simulink model "d_024"  (Simulink 5.1)
settings: Solver=ode45  StartTime=0.0  StopTime=10.0  RelTol=1e-3
libraries: fm_lib x37
settings Model: Creator=fmilano  LastModifiedBy=fmilano  ExtModeAutoUpdateStatusClock=off  SignalLoggingName=logsout  BooleanDataType=on  RTWOptions="-aEnforceIntegerDowncast=1 -aFoldNonRolledExpr=1 -aInlineInvariantSignals=1 -aInlineParameters=0 -aLocalBlockOutputs=1 -aRollThreshold=5 -aZeroInternalMemoryAtStartup=1 -aZeroExternalMemoryAtStartup=1 -aInitFltsAndDblsToZero=1 -aForceBlockIOInitOptimize=0 -aGenerateReport=0 -aGenCodeOnly=0 -aRTWVerbose=1 -aIncludeHyperlinkInReport=0 -aLaunchReport=0 -aGenerateTraceInfo=0  -aForceParamTrailComments=0 -aGenerateComments=1 -aIgnoreCustomStorageClasses=1 -aIncHierarchyInIds=0 -aMaxRTWIdLen=31 -aShowEliminatedStatements=0 -aIncDataTypeInIds=0 -aInsertBlockDesc=0 -aIgnoreTestpoints=0 -aSimulinkBlockComments=1 -aInlinedPrmAccess=\"Literals\"  -aSuppressErrorStatus=0 -aModelReferenceCompliant=1 -aParenthesesLevel=\"Nominal\" -aModelStepFunctionPrototypeControlCompliant=0 -aPortableWordSizes=0 -aParMdlRefBuildCompliant=1 -aSupportNonInlinedSFcns=1 -aSupportContinuousTime=1 -aSupportComplex=1 -aSupportNonFinite=1 -aSupportAbsoluteTime=1 -aMultiwordLength=2048 -aTargetPreCompLibLocation=\"\" -aTargetLibSuffix=\"\" -aTargetFunctionLibrary=\"ANSI_C\" -aTargetFcnLib=\"ansi_tfl_tmw.mat\" -aMultiInstanceERTCode=0 -aLogVarNameModifier=\"rt_\" -aERTFirstTimeCompliant=0 -aIsPILTarget=0 -aCombineOutputUpdateFcns=0 -aGenerateASAP2=0 -aGenerateClassInterface=0 -aGenerateTestInterfaces=0 -aGenerateSampleERTMain=0 -aGenerateFullHeader=1 -aUtilityFuncGeneration=\"Auto\" -aIncludeFileDelimiter=\"Auto\" -aIncludeMdlTerminateFcn=1 -aPurelyIntegerCode=0 -aAutosarCompliant=0 -aERTCustomFileBanners=0 -aRTWCAPIStates=0 -aRTWCAPIParams=0 -aRTWCAPISignals=0 -aMatFileLogging=1 -aCompOptLevelCompliant=0 -aCPPClassGenCompliant=0 -aExtModeIntrfLevel=\"Level1\" -aExtModeMexFile=\"ext_comm\" -aExtModeTransport=0 -aExtModeStaticAllocSize=1000000 -aExtModeTesting=0 -aExtModeStaticAlloc=0 -aExtMode=0 -aERTMultiwordLength=256 -aERTMultiwordTypeDef=\"System defined\"  -aGenerateTraceInfo=0 -aGenerateTraceInfo=0 -aGenerateTraceInfo=0 -aGenerateTraceInfo=0 -aPrefixModelToSubsysFcnNames=1"

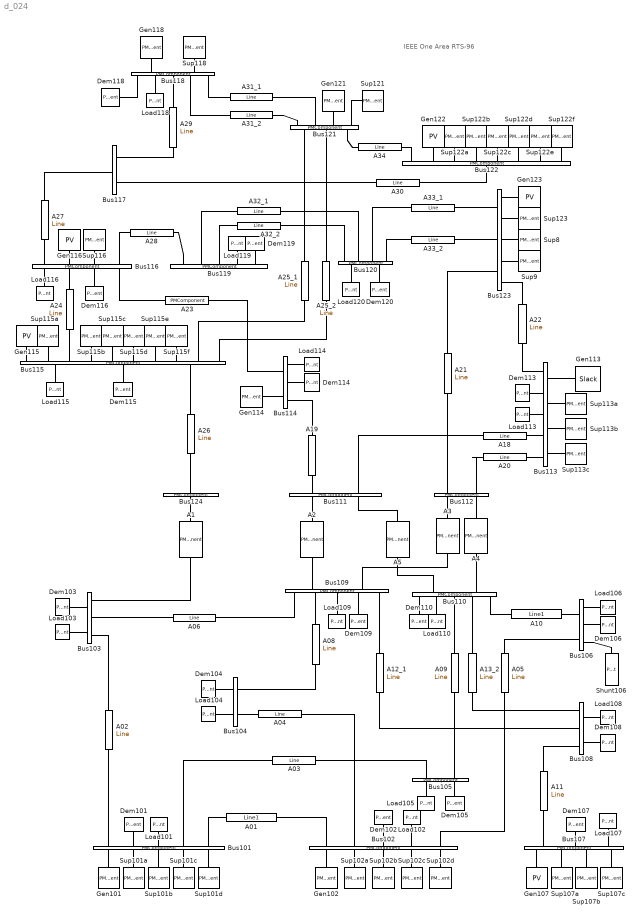
== system d_024 ==
  note: IEEE One Area RTS-96
  A01 : fm_lib/Power Flow/Line1  Tag=PSATblock  Description=Power Flow  PhysicalDomain=psatdomain  SubClassName=unknown  LeftPortType=p1  RightPortType=p1  LConnTagsString=__newl0  RConnTagsString=__newr0  p3_4_5q="[100  138  60]"  p6q=0  p8q=0.0026  p9q=0.0139  p10q=0.4611  p13_14_15q="[1.93  0.0  2.00]"  p16q=on
  A02 : fm_lib/Power Flow/Line  Tag=PSATblock  Description=Power Flow  Orientation=up  PhysicalDomain=psatdomain  SubClassName=unknown  LeftPortType=p1  RightPortType=p1  LConnTagsString=__newl0  RConnTagsString=__newr0  p3_4_5q="[100  138  60]"  p6q=0  p8q=0.0546  p9q=0.2112  p10q=0.0572  p13_14_15q="[2.08  0.0  2.20]"  p16q=on
  A03 : fm_lib/Power Flow/Line  Tag=PSATblock  Description=Power Flow  PhysicalDomain=psatdomain  SubClassName=unknown  LeftPortType=p1  RightPortType=p1  LConnTagsString=__newl0  RConnTagsString=__newr0  p3_4_5q="[100  138  60]"  p6q=0  p8q=0.0218  p9q=0.0845  p10q=0.0229  p13_14_15q="[2.08  0.0  2.20]"  p16q=on
  A04 : fm_lib/Power Flow/Line  Tag=PSATblock  Description=Power Flow  Orientation=left  PhysicalDomain=psatdomain  SubClassName=unknown  LeftPortType=p1  RightPortType=p1  LConnTagsString=__newl0  RConnTagsString=__newr0  p3_4_5q="[100  138  60]"  p6q=0  p8q=0.0328  p9q=0.1267  p10q=0.0343  p13_14_15q="[2.08  0.0  2.20]"  p16q=on
  A05 : fm_lib/Power Flow/Line  Tag=PSATblock  Description=Power Flow  Orientation=up  PhysicalDomain=psatdomain  SubClassName=unknown  LeftPortType=p1  RightPortType=p1  LConnTagsString=__newl0  RConnTagsString=__newr0  p3_4_5q="[100  138  60]"  p6q=0  p8q=0.0497  p9q=0.192  p10q=0.052  p13_14_15q="[2.08  0.0  2.20]"  p16q=on
  A06 : fm_lib/Power Flow/Line  Tag=PSATblock  Description=Power Flow  Orientation=left  PhysicalDomain=psatdomain  SubClassName=unknown  LeftPortType=p1  RightPortType=p1  LConnTagsString=__newl0  RConnTagsString=__newr0  p3_4_5q="[100  138  60]"  p6q=0  p8q=0.0308  p9q=0.119  p10q=0.0322  p13_14_15q="[2.08  0.0  2.20]"  p16q=on
  A08 : fm_lib/Power Flow/Line  Tag=PSATblock  Description=Power Flow  Orientation=down  PhysicalDomain=psatdomain  SubClassName=unknown  LeftPortType=p1  RightPortType=p1  LConnTagsString=__newl0  RConnTagsString=__newr0  p3_4_5q="[100  138  60]"  p6q=0  p8q=0.0268  p9q=0.1037  p10q=0.0281  p13_14_15q="[2.08  0.0  2.20]"  p16q=on
  A09 : fm_lib/Power Flow/Line  Tag=PSATblock  Description=Power Flow  Orientation=down  PhysicalDomain=psatdomain  SubClassName=unknown  LeftPortType=p1  RightPortType=p1  LConnTagsString=__newl0  RConnTagsString=__newr0  p3_4_5q="[100  138  60]"  p6q=0  p8q=0.0228  p9q=0.0883  p10q=0.0239  p13_14_15q="[2.08  0.0  2.20]"  p16q=on
  A1 : PMComponent  Tag=PSATblock  Description=Power Flow  Orientation=up  PhysicalDomain=psatdomain  LeftPortType=p1  RightPortType=p1  LConnTagsString=__newl0  RConnTagsString=__newr0  mask(Line){p3_4_5q=[100  138  60], p7q=138/230, p8q=0.0023, p9q=0.0839, p11q=1.015, p13_14_15q=[5.10  0.0  6.00], p16q=on}
      mask prompts: p3_4_5q "Power, Voltage and Frequency Ratings [MVA, kV, Hz]"; p7q "Primary and secondary voltage ratio [kV/kV]"; p8q "Resistance [p.u.]"; p9q "Reactance [p.u.]"; p11q "Fixed tap ratio [p.u./p.u.]"; p13_14_15q "Imax, Pmax and Smax  [p.u., p.u., p.u.]"; p16q "Connected"
      mask help: This block defines a transformer with constant tap ratio.
      mask init:
      | [x,y] = fm_draw('circle');
      | [x2,y2] = fm_draw('2');
      mask CallbackString: ||||||fm_block
      mask Display:
      | plot(x,y,x+1.4,y,[-1 -1.3],[0 0],[2.4 2.7],[0 0])
      | color('green')
      | plot([-0.8 0.7],[-1.2 1.2],[0.5 0.7],[1.1 1.2],[0.7 0.7],[1.0 1.2])
      | plot(1.5+0.65*x2,0.65*y2)
  A10 : fm_lib/Power Flow/Line1  Tag=PSATblock  Description=Power Flow  PhysicalDomain=psatdomain  SubClassName=unknown  LeftPortType=p1  RightPortType=p1  LConnTagsString=__newl0  RConnTagsString=__newr0  p3_4_5q="[100  138  60]"  p6q=0  p8q=0.0139  p9q=0.0605  p10q=2.459  p13_14_15q="[1.93  0.0  2.00]"  p16q=on
  A11 : fm_lib/Power Flow/Line  Tag=PSATblock  Description=Power Flow  Orientation=up  PhysicalDomain=psatdomain  SubClassName=unknown  LeftPortType=p1  RightPortType=p1  LConnTagsString=__newl0  RConnTagsString=__newr0  p3_4_5q="[100  138  60]"  p6q=0  p8q=0.0159  p9q=0.0614  p10q=0.0166  p13_14_15q="[2.08  0.0  2.20]"  p16q=on
  A12_1 : fm_lib/Power Flow/Line  Tag=PSATblock  Description=Power Flow  Orientation=down  PhysicalDomain=psatdomain  SubClassName=unknown  LeftPortType=p1  RightPortType=p1  LConnTagsString=__newl0  RConnTagsString=__newr0  p3_4_5q="[100  138  60]"  p6q=0  p8q=0.0427  p9q=0.1651  p10q=0.0447  p13_14_15q="[2.08  0.0  2.20]"  p16q=on
  A13_2 : fm_lib/Power Flow/Line  Tag=PSATblock  Description=Power Flow  Orientation=down  PhysicalDomain=psatdomain  SubClassName=unknown  LeftPortType=p1  RightPortType=p1  LConnTagsString=__newl0  RConnTagsString=__newr0  p3_4_5q="[100  138  60]"  p6q=0  p8q=0.0427  p9q=0.1651  p10q=0.0447  p13_14_15q="[2.08  0.0  2.20]"  p16q=on
  A18 : fm_lib/Power Flow/Line  Tag=PSATblock  Description=Power Flow  Orientation=left  PhysicalDomain=psatdomain  SubClassName=unknown  LeftPortType=p1  RightPortType=p1  LConnTagsString=__newl0  RConnTagsString=__newr0  p3_4_5q="[100  230  60]"  p6q=0  p8q=0.006  p9q=0.048  p10q=0.100  p13_14_15q="[6.00  0.0  6.25]"  p16q=on
  A19 : PMComponent  Tag=PSATblock  Description=Power Flow  Orientation=down  PhysicalDomain=psatdomain  LeftPortType=p1  RightPortType=p1  LConnTagsString=__newl0  RConnTagsString=__newr0  mask(Line){p3_4_5q=[100  230  60], p6q=0, p8q=0.0054, p9q=0.0418, p10q=0.0879, p13_14_15q=[6.00  0.0  6.25], p16q=on}
      mask prompts: p3_4_5q "Power, Voltage and Frequency Ratings [MVA, kV, Hz]"; p6q "Length of line [km] (0 for p.u. parameters)"; p8q "Resistance [p.u. (Ohms/km)]"; p9q "Reactance [p.u. (H/km)]"; p10q "Susceptance [p.u. (F/km)]"; p13_14_15q "Imax, Pmax and Smax [p.u., p.u., p.u.]"; p16q "Connected"
      mask help: This block defines a pi model for a tree phase line.
      mask init:
      | [xp,yp] = fm_draw('pi');
      mask CallbackString: ||||||fm_block
      mask Display:
      | plot([-1  1  1 -1 -1],[-0.2 -0.2 0.2 0.2 -0.2])
      | color('blue')
      | plot(0.35*xp,0.2*yp)
  A2 : PMComponent  Tag=PSATblock  Description=Power Flow  Orientation=up  PhysicalDomain=psatdomain  LeftPortType=p1  RightPortType=p1  LConnTagsString=__newl0  RConnTagsString=__newr0  mask(Line){p3_4_5q=[100  138  60], p7q=138/230, p8q=0.0023, p9q=0.0839, p11q=1.03, p13_14_15q=[5.10  0.0  6.00], p16q=on}
      mask prompts: p3_4_5q "Power, Voltage and Frequency Ratings [MVA, kV, Hz]"; p7q "Primary and secondary voltage ratio [kV/kV]"; p8q "Resistance [p.u.]"; p9q "Reactance [p.u.]"; p11q "Fixed tap ratio [p.u./p.u.]"; p13_14_15q "Imax, Pmax and Smax  [p.u., p.u., p.u.]"; p16q "Connected"
      mask help: This block defines a transformer with constant tap ratio.
      mask init:
      | [x,y] = fm_draw('circle');
      | [x2,y2] = fm_draw('2');
      mask CallbackString: ||||||fm_block
      mask Display:
      | plot(x,y,x+1.4,y,[-1 -1.3],[0 0],[2.4 2.7],[0 0])
      | color('green')
      | plot([-0.8 0.7],[-1.2 1.2],[0.5 0.7],[1.1 1.2],[0.7 0.7],[1.0 1.2])
      | plot(1.5+0.65*x2,0.65*y2)
  A20 : fm_lib/Power Flow/Line  Tag=PSATblock  Description=Power Flow  Orientation=left  PhysicalDomain=psatdomain  SubClassName=unknown  LeftPortType=p1  RightPortType=p1  LConnTagsString=__newl0  RConnTagsString=__newr0  p3_4_5q="[100  230  60]"  p6q=0  p8q=0.006  p9q=0.048  p10q=0.100  p13_14_15q="[6.00  0.0  6.25]"  p16q=on
  A21 : fm_lib/Power Flow/Line  Tag=PSATblock  Description=Power Flow  Orientation=down  PhysicalDomain=psatdomain  SubClassName=unknown  LeftPortType=p1  RightPortType=p1  LConnTagsString=__newl0  RConnTagsString=__newr0  p3_4_5q="[100  230  60]"  p6q=0  p8q=0.0124  p9q=0.0966  p10q=0.203  p13_14_15q="[6.00  0.0  6.25]"  p16q=on
  A22 : fm_lib/Power Flow/Line  Tag=PSATblock  Description=Power Flow  Orientation=up  PhysicalDomain=psatdomain  SubClassName=unknown  LeftPortType=p1  RightPortType=p1  LConnTagsString=__newl0  RConnTagsString=__newr0  p3_4_5q="[100  230  60]"  p6q=0  p8q=0.0111  p9q=0.0865  p10q=0.1818  p13_14_15q="[6.00  0.0  6.25]"  p16q=on
  A23 : PMComponent  Tag=PSATblock  Description=Power Flow  PhysicalDomain=psatdomain  LeftPortType=p1  RightPortType=p1  LConnTagsString=__newl0  RConnTagsString=__newr0  mask(Line){p3_4_5q=[100  230  60], p6q=0, p8q=0.005, p9q=0.0589, p10q=0.0818, p13_14_15q=[6.00  0.0  6.25], p16q=on}
      mask prompts: p3_4_5q "Power, Voltage and Frequency Ratings [MVA, kV, Hz]"; p6q "Length of line [km] (0 for p.u. parameters)"; p8q "Resistance [p.u. (Ohms/km)]"; p9q "Reactance [p.u. (H/km)]"; p10q "Susceptance [p.u. (F/km)]"; p13_14_15q "Imax, Pmax and Smax [p.u., p.u., p.u.]"; p16q "Connected"
      mask help: This block defines a pi model for a tree phase line.
      mask init:
      | [xp,yp] = fm_draw('pi');
      mask CallbackString: ||||||fm_block
      mask Display:
      | plot([-1  1  1 -1 -1],[-0.2 -0.2 0.2 0.2 -0.2])
      | color('blue')
      | plot(0.35*xp,0.2*yp)
  A24 : fm_lib/Power Flow/Line  Tag=PSATblock  Description=Power Flow  Orientation=down  PhysicalDomain=psatdomain  SubClassName=unknown  LeftPortType=p1  RightPortType=p1  LConnTagsString=__newl0  RConnTagsString=__newr0  p3_4_5q="[100  230  60]"  p6q=0  p8q=0.0022  p9q=0.0173  p10q=0.0364  p13_14_15q="[6.00  0.0  6.25]"  p16q=on
  A25_1 : fm_lib/Power Flow/Line  Tag=PSATblock  Description=Power Flow  Orientation=down  PhysicalDomain=psatdomain  SubClassName=unknown  LeftPortType=p1  RightPortType=p1  LConnTagsString=__newl0  RConnTagsString=__newr0  p3_4_5q="[100  230  60]"  p6q=0  p8q=0.0063  p9q=0.049  p10q=0.103  p13_14_15q="[6.00  0.0  6.25]"  p16q=on
  A25_2 : fm_lib/Power Flow/Line  Tag=PSATblock  Description=Power Flow  Orientation=down  PhysicalDomain=psatdomain  SubClassName=unknown  LeftPortType=p1  RightPortType=p1  LConnTagsString=__newl0  RConnTagsString=__newr0  p3_4_5q="[100  230  60]"  p6q=0  p8q=0.0063  p9q=0.049  p10q=0.103  p13_14_15q="[6.00  0.0  6.25]"  p16q=on
  A26 : fm_lib/Power Flow/Line  Tag=PSATblock  Description=Power Flow  Orientation=down  PhysicalDomain=psatdomain  SubClassName=unknown  LeftPortType=p1  RightPortType=p1  LConnTagsString=__newl0  RConnTagsString=__newr0  p3_4_5q="[100  230  60]"  p6q=0  p8q=0.0067  p9q=0.0519  p10q=0.1091  p13_14_15q="[6.00  0.0  6.25]"  p16q=on
  A27 : fm_lib/Power Flow/Line  Tag=PSATblock  Description=Power Flow  Orientation=down  PhysicalDomain=psatdomain  SubClassName=unknown  LeftPortType=p1  RightPortType=p1  LConnTagsString=__newl0  RConnTagsString=__newr0  p3_4_5q="[100  230  60]"  p6q=0  p8q=0.003  p9q=0.0259  p10q=0.0545  p13_14_15q="[6.00  0.0  6.25]"  p16q=on
  A28 : fm_lib/Power Flow/Line  Tag=PSATblock  Description=Power Flow  Orientation=left  PhysicalDomain=psatdomain  SubClassName=unknown  LeftPortType=p1  RightPortType=p1  LConnTagsString=__newl0  RConnTagsString=__newr0  p3_4_5q="[100  230  60]"  p6q=0  p8q=0.003  p9q=0.0231  p10q=0.0485  p13_14_15q="[6.00  0.0  6.25]"  p16q=on
  A29 : fm_lib/Power Flow/Line  Tag=PSATblock  Description=Power Flow  Orientation=down  PhysicalDomain=psatdomain  SubClassName=unknown  LeftPortType=p1  RightPortType=p1  LConnTagsString=__newl0  RConnTagsString=__newr0  p3_4_5q="[100  230  60]"  p6q=0  p8q=0.0018  p9q=0.0144  p10q=0.0303  p13_14_15q="[6.00  0.0  6.25]"  p16q=on
  A3 : PMComponent  Tag=PSATblock  Description=Power Flow  Orientation=up  PhysicalDomain=psatdomain  LeftPortType=p1  RightPortType=p1  LConnTagsString=__newl0  RConnTagsString=__newr0  mask(Line){p3_4_5q=[100  138  60], p7q=138/230, p8q=0.0023, p9q=0.0839, p11q=1.03, p13_14_15q=[5.10  0.0  6.00], p16q=on}
      mask prompts: p3_4_5q "Power, Voltage and Frequency Ratings [MVA, kV, Hz]"; p7q "Primary and secondary voltage ratio [kV/kV]"; p8q "Resistance [p.u.]"; p9q "Reactance [p.u.]"; p11q "Fixed tap ratio [p.u./p.u.]"; p13_14_15q "Imax, Pmax and Smax  [p.u., p.u., p.u.]"; p16q "Connected"
      mask help: This block defines a transformer with constant tap ratio.
      mask init:
      | [x,y] = fm_draw('circle');
      | [x2,y2] = fm_draw('2');
      mask CallbackString: ||||||fm_block
      mask Display:
      | plot(x,y,x+1.4,y,[-1 -1.3],[0 0],[2.4 2.7],[0 0])
      | color('green')
      | plot([-0.8 0.7],[-1.2 1.2],[0.5 0.7],[1.1 1.2],[0.7 0.7],[1.0 1.2])
      | plot(1.5+0.65*x2,0.65*y2)
  A30 : fm_lib/Power Flow/Line  Tag=PSATblock  Description=Power Flow  Orientation=left  PhysicalDomain=psatdomain  SubClassName=unknown  LeftPortType=p1  RightPortType=p1  LConnTagsString=__newl0  RConnTagsString=__newr0  p3_4_5q="[100  230  60]"  p6q=0  p8q=0.0135  p9q=0.1053  p10q=0.2212  p13_14_15q="[6.00  0.0  6.25]"  p16q=on
  A31_1 : fm_lib/Power Flow/Line  Tag=PSATblock  Description=Power Flow  PhysicalDomain=psatdomain  SubClassName=unknown  LeftPortType=p1  RightPortType=p1  LConnTagsString=__newl0  RConnTagsString=__newr0  p3_4_5q="[100  230  60]"  p6q=0  p8q=0.0033  p9q=0.0269  p10q=0.0545  p13_14_15q="[6.00  0.0  6.25]"  p16q=on
  A31_2 : fm_lib/Power Flow/Line  Tag=PSATblock  Description=Power Flow  PhysicalDomain=psatdomain  SubClassName=unknown  LeftPortType=p1  RightPortType=p1  LConnTagsString=__newl0  RConnTagsString=__newr0  p3_4_5q="[100  230  60]"  p6q=0  p8q=0.0033  p9q=0.0269  p10q=0.0545  p13_14_15q="[6.00  0.0  6.25]"  p16q=on
  A32_1 : fm_lib/Power Flow/Line  Tag=PSATblock  Description=Power Flow  PhysicalDomain=psatdomain  SubClassName=unknown  LeftPortType=p1  RightPortType=p1  LConnTagsString=__newl0  RConnTagsString=__newr0  p3_4_5q="[100  230  60]"  p6q=0  p8q=0.0051  p9q=0.0396  p10q=0.0833  p13_14_15q="[6.00  0.0  6.25]"  p16q=on
  A32_2 : fm_lib/Power Flow/Line  Tag=PSATblock  Description=Power Flow  PhysicalDomain=psatdomain  SubClassName=unknown  LeftPortType=p1  RightPortType=p1  LConnTagsString=__newl0  RConnTagsString=__newr0  p3_4_5q="[100  230  60]"  p6q=0  p8q=0.0051  p9q=0.0396  p10q=0.0833  p13_14_15q="[6.00  0.0  6.25]"  p16q=on
  A33_1 : fm_lib/Power Flow/Line  Tag=PSATblock  Description=Power Flow  Orientation=left  PhysicalDomain=psatdomain  SubClassName=unknown  LeftPortType=p1  RightPortType=p1  LConnTagsString=__newl0  RConnTagsString=__newr0  p3_4_5q="[100  230  60]"  p6q=0  p8q=0.0028  p9q=0.0216  p10q=0.0455  p13_14_15q="[6.00  0.0  6.25]"  p16q=on
  A33_2 : fm_lib/Power Flow/Line  Tag=PSATblock  Description=Power Flow  Orientation=left  PhysicalDomain=psatdomain  SubClassName=unknown  LeftPortType=p1  RightPortType=p1  LConnTagsString=__newl0  RConnTagsString=__newr0  p3_4_5q="[100  230  60]"  p6q=0  p8q=0.0028  p9q=0.0216  p10q=0.0455  p13_14_15q="[6.00  0.0  6.25]"  p16q=on
  A34 : fm_lib/Power Flow/Line  Tag=PSATblock  Description=Power Flow  PhysicalDomain=psatdomain  SubClassName=unknown  LeftPortType=p1  RightPortType=p1  LConnTagsString=__newl0  RConnTagsString=__newr0  p3_4_5q="[100  230  60]"  p6q=0  p8q=0.0087  p9q=0.0678  p10q=0.1424  p13_14_15q="[6.00  0.0  6.25]"  p16q=on
  A4 : PMComponent  Tag=PSATblock  Description=Power Flow  Orientation=up  PhysicalDomain=psatdomain  LeftPortType=p1  RightPortType=p1  LConnTagsString=__newl0  RConnTagsString=__newr0  mask(Line){p3_4_5q=[100  138  60], p7q=138/230, p8q=0.0023, p9q=0.0839, p11q=1.015, p13_14_15q=[5.10  0.0  6.00], p16q=on}
      mask prompts: p3_4_5q "Power, Voltage and Frequency Ratings [MVA, kV, Hz]"; p7q "Primary and secondary voltage ratio [kV/kV]"; p8q "Resistance [p.u.]"; p9q "Reactance [p.u.]"; p11q "Fixed tap ratio [p.u./p.u.]"; p13_14_15q "Imax, Pmax and Smax  [p.u., p.u., p.u.]"; p16q "Connected"
      mask help: This block defines a transformer with constant tap ratio.
      mask init:
      | [x,y] = fm_draw('circle');
      | [x2,y2] = fm_draw('2');
      mask CallbackString: ||||||fm_block
      mask Display:
      | plot(x,y,x+1.4,y,[-1 -1.3],[0 0],[2.4 2.7],[0 0])
      | color('green')
      | plot([-0.8 0.7],[-1.2 1.2],[0.5 0.7],[1.1 1.2],[0.7 0.7],[1.0 1.2])
      | plot(1.5+0.65*x2,0.65*y2)
  A5 : PMComponent  Tag=PSATblock  Description=Power Flow  Orientation=up  PhysicalDomain=psatdomain  LeftPortType=p1  RightPortType=p1  LConnTagsString=__newl0  RConnTagsString=__newr0  mask(Line){p3_4_5q=[100  138  60], p7q=138/230, p8q=0.0023, p9q=0.0839, p11q=1.015, p13_14_15q=[5.10  0.0  6.00], p16q=on}
      mask prompts: p3_4_5q "Power, Voltage and Frequency Ratings [MVA, kV, Hz]"; p7q "Primary and secondary voltage ratio [kV/kV]"; p8q "Resistance [p.u.]"; p9q "Reactance [p.u.]"; p11q "Fixed tap ratio [p.u./p.u.]"; p13_14_15q "Imax, Pmax and Smax  [p.u., p.u., p.u.]"; p16q "Connected"
      mask help: This block defines a transformer with constant tap ratio.
      mask init:
      | [x,y] = fm_draw('circle');
      | [x2,y2] = fm_draw('2');
      mask CallbackString: ||||||fm_block
      mask Display:
      | plot(x,y,x+1.4,y,[-1 -1.3],[0 0],[2.4 2.7],[0 0])
      | color('green')
      | plot([-0.8 0.7],[-1.2 1.2],[0.5 0.7],[1.1 1.2],[0.7 0.7],[1.0 1.2])
      | plot(1.5+0.65*x2,0.65*y2)
  Bus101 : PMComponent  Tag=PSATblock  Description=Connection  Orientation=up  PhysicalDomain=psatdomain  LeftPortType=p1  RightPortType=p1  LConnTagsString=__newl0|__newl1|__newl2|__newl3|__newl4  RConnTagsString=__newr0|__newr1|__newr2|__newr3|__newr4  mask(Bus){in=5, out=5, p2q=138, p3_4q=[1.00  0.00], p5q=2, p6q=1}
      mask prompts: in "Number of inputs:"; out "Number of outputs:"; p2q "Voltage Rating [kV]"; p3_4q "Voltage initial guess [p.u.  rad]"; p5q "Area number"; p6q "Region number"
      mask help: Bus block.
      mask init:
      | fm_inout
      mask CallbackString: ||||fm_block|
      mask Display: plot([0 1 1 0 0],[0 0 1 1 0])
  Bus102 : PMComponent  Tag=PSATblock  Description=Connection  Orientation=up  PhysicalDomain=psatdomain  LeftPortType=p1  RightPortType=p1  LConnTagsString=__newl0|__newl1|__newl2|__newl3|__newl4  RConnTagsString=__newr0|__newr1|__newr2|__newr3|__newr4  mask(Bus){in=5, out=5, p2q=138, p3_4q=[1.00  0.00], p5q=2, p6q=1}
      mask prompts: in "Number of inputs:"; out "Number of outputs:"; p2q "Voltage Rating [kV]"; p3_4q "Voltage initial guess [p.u.  rad]"; p5q "Area number"; p6q "Region number"
      mask help: Bus block.
      mask init:
      | fm_inout
      mask CallbackString: ||||fm_block|
      mask Display: plot([0 1 1 0 0],[0 0 1 1 0])
  Bus103 : PMComponent  Tag=PSATblock  Description=Connection  Orientation=left  PhysicalDomain=psatdomain  LeftPortType=p1  RightPortType=p1  LConnTagsString=__newl0|__newl1|__newl2  RConnTagsString=__newr0|__newr1  mask(Bus){in=3, out=2, p2q=138, p3_4q=[1.00   0.00], p5q=2, p6q=1}
      mask prompts: in "Number of inputs:"; out "Number of outputs:"; p2q "Voltage Rating [kV]"; p3_4q "Voltage initial guess [p.u.  rad]"; p5q "Area number"; p6q "Region number"
      mask help: Bus block.
      mask init:
      | fm_inout
      mask CallbackString: ||||fm_block|
      mask Display: plot([0 1 1 0 0],[0 0 1 1 0])
  Bus104 : PMComponent  Tag=PSATblock  Description=Connection  Orientation=left  PhysicalDomain=psatdomain  LeftPortType=p1  RightPortType=p1  LConnTagsString=__newl0|__newl1  RConnTagsString=__newr0|__newr1  mask(Bus){in=2, out=2, p2q=138, p3_4q=[1.00   0.00], p5q=2, p6q=1}
      mask prompts: in "Number of inputs:"; out "Number of outputs:"; p2q "Voltage Rating [kV]"; p3_4q "Voltage initial guess [p.u.  rad]"; p5q "Area number"; p6q "Region number"
      mask help: Bus block.
      mask init:
      | fm_inout
      mask CallbackString: ||||fm_block|
      mask Display: plot([0 1 1 0 0],[0 0 1 1 0])
  Bus105 : PMComponent  Tag=PSATblock  Description=Connection  Orientation=down  PhysicalDomain=psatdomain  LeftPortType=p1  RightPortType=p1  LConnTagsString=__newl0|__newl1  RConnTagsString=__newr0|__newr1  mask(Bus){in=2, out=2, p2q=138, p3_4q=[1.00   0.00], p5q=2, p6q=1}
      mask prompts: in "Number of inputs:"; out "Number of outputs:"; p2q "Voltage Rating [kV]"; p3_4q "Voltage initial guess [p.u.  rad]"; p5q "Area number"; p6q "Region number"
      mask help: Bus block.
      mask init:
      | fm_inout
      mask CallbackString: ||||fm_block|
      mask Display: plot([0 1 1 0 0],[0 0 1 1 0])
  Bus106 : PMComponent  Tag=PSATblock  Description=Connection  PhysicalDomain=psatdomain  LeftPortType=p1  RightPortType=p1  LConnTagsString=__newl0|__newl1  RConnTagsString=__newr0|__newr1|__newr2  mask(Bus){in=2, out=3, p2q=138, p3_4q=[1.00   0.00], p5q=2, p6q=1}
      mask prompts: in "Number of inputs:"; out "Number of outputs:"; p2q "Voltage Rating [kV]"; p3_4q "Voltage initial guess [p.u.  rad]"; p5q "Area number"; p6q "Region number"
      mask help: Bus block.
      mask init:
      | fm_inout
      mask CallbackString: ||||fm_block|
      mask Display: plot([0 1 1 0 0],[0 0 1 1 0])
  Bus107 : PMComponent  Tag=PSATblock  Description=Connection  Orientation=up  PhysicalDomain=psatdomain  LeftPortType=p1  RightPortType=p1  LConnTagsString=__newl0|__newl1|__newl2|__newl3  RConnTagsString=__newr0|__newr1|__newr2  mask(Bus){in=4, out=3, p2q=138, p3_4q=[1.00  0.00], p5q=2, p6q=1}
      mask prompts: in "Number of inputs:"; out "Number of outputs:"; p2q "Voltage Rating [kV]"; p3_4q "Voltage initial guess [p.u.  rad]"; p5q "Area number"; p6q "Region number"
      mask help: Bus block.
      mask init:
      | fm_inout
      mask CallbackString: ||||fm_block|
      mask Display: plot([0 1 1 0 0],[0 0 1 1 0])
  Bus108 : PMComponent  Tag=PSATblock  Description=Connection  PhysicalDomain=psatdomain  LeftPortType=p1  RightPortType=p1  LConnTagsString=__newl0|__newl1|__newl2  RConnTagsString=__newr0|__newr1  mask(Bus){in=3, out=2, p2q=138, p3_4q=[1.00   0.00], p5q=2, p6q=1}
      mask prompts: in "Number of inputs:"; out "Number of outputs:"; p2q "Voltage Rating [kV]"; p3_4q "Voltage initial guess [p.u.  rad]"; p5q "Area number"; p6q "Region number"
      mask help: Bus block.
      mask init:
      | fm_inout
      mask CallbackString: ||||fm_block|
      mask Display: plot([0 1 1 0 0],[0 0 1 1 0])
  Bus109 : PMComponent  Tag=PSATblock  Description=Connection  Orientation=down  PhysicalDomain=psatdomain  LeftPortType=p1  RightPortType=p1  LConnTagsString=__newl0|__newl1  RConnTagsString=__newr0|__newr1|__newr2|__newr3|__newr4  mask(Bus){in=2, out=5, p2q=138, p3_4q=[1.00  0.00], p5q=2, p6q=1}
      mask prompts: in "Number of inputs:"; out "Number of outputs:"; p2q "Voltage Rating [kV]"; p3_4q "Voltage initial guess [p.u.  rad]"; p5q "Area number"; p6q "Region number"
      mask help: Bus block.
      mask init:
      | fm_inout
      mask CallbackString: ||||fm_block|
      mask Display: plot([0 1 1 0 0],[0 0 1 1 0])
  Bus110 : PMComponent  Tag=PSATblock  Description=Connection  Orientation=down  PhysicalDomain=psatdomain  LeftPortType=p1  RightPortType=p1  LConnTagsString=__newl0|__newl1  RConnTagsString=__newr0|__newr1|__newr2|__newr3|__newr4  mask(Bus){in=2, out=5, p2q=138, p3_4q=[1.00  0.00], p5q=2, p6q=1}
      mask prompts: in "Number of inputs:"; out "Number of outputs:"; p2q "Voltage Rating [kV]"; p3_4q "Voltage initial guess [p.u.  rad]"; p5q "Area number"; p6q "Region number"
      mask help: Bus block.
      mask init:
      | fm_inout
      mask CallbackString: ||||fm_block|
      mask Display: plot([0 1 1 0 0],[0 0 1 1 0])
  Bus111 : PMComponent  Tag=PSATblock  Description=Connection  Orientation=down  PhysicalDomain=psatdomain  LeftPortType=p1  RightPortType=p1  LConnTagsString=__newl0|__newl1  RConnTagsString=__newr0|__newr1  mask(Bus){in=2, out=2, p2q=230, p3_4q=[1.00  0.00], p5q=3, p6q=1}
      mask prompts: in "Number of inputs:"; out "Number of outputs:"; p2q "Voltage Rating [kV]"; p3_4q "Voltage initial guess [p.u.  rad]"; p5q "Area number"; p6q "Region number"
      mask help: Bus block.
      mask init:
      | fm_inout
      mask CallbackString: ||||fm_block|
      mask Display: plot([0 1 1 0 0],[0 0 1 1 0])
  Bus112 : PMComponent  Tag=PSATblock  Description=Connection  Orientation=down  PhysicalDomain=psatdomain  LeftPortType=p1  RightPortType=p1  LConnTagsString=__newl0|__newl1  RConnTagsString=__newr0|__newr1  mask(Bus){in=2, out=2, p2q=230, p3_4q=[1.00  0.00], p5q=3, p6q=1}
      mask prompts: in "Number of inputs:"; out "Number of outputs:"; p2q "Voltage Rating [kV]"; p3_4q "Voltage initial guess [p.u.  rad]"; p5q "Area number"; p6q "Region number"
      mask help: Bus block.
      mask init:
      | fm_inout
      mask CallbackString: ||||fm_block|
      mask Display: plot([0 1 1 0 0],[0 0 1 1 0])
  Bus113 : PMComponent  Tag=PSATblock  Description=Connection  Orientation=left  PhysicalDomain=psatdomain  LeftPortType=p1  RightPortType=p1  LConnTagsString=__newl0|__newl1|__newl2|__newl3  RConnTagsString=__newr0|__newr1|__newr2|__newr3|__newr4  mask(Bus){in=4, out=5, p2q=230, p3_4q=[1.00   0.00], p5q=3, p6q=1}
      mask prompts: in "Number of inputs:"; out "Number of outputs:"; p2q "Voltage Rating [kV]"; p3_4q "Voltage initial guess [p.u.  rad]"; p5q "Area number"; p6q "Region number"
      mask help: Bus block.
      mask init:
      | fm_inout
      mask CallbackString: ||||fm_block|
      mask Display: plot([0 1 1 0 0],[0 0 1 1 0])
  Bus114 : PMComponent  Tag=PSATblock  Description=Connection  PhysicalDomain=psatdomain  LeftPortType=p1  RightPortType=p1  LConnTagsString=__newl0|__newl1  RConnTagsString=__newr0|__newr1|__newr2  mask(Bus){in=2, out=3, p2q=230, p3_4q=[1.00   0.00], p5q=3, p6q=1}
      mask prompts: in "Number of inputs:"; out "Number of outputs:"; p2q "Voltage Rating [kV]"; p3_4q "Voltage initial guess [p.u.  rad]"; p5q "Area number"; p6q "Region number"
      mask help: Bus block.
      mask init:
      | fm_inout
      mask CallbackString: ||||fm_block|
      mask Display: plot([0 1 1 0 0],[0 0 1 1 0])
  Bus115 : PMComponent  Tag=PSATblock  Description=Connection  Orientation=down  PhysicalDomain=psatdomain  LeftPortType=p1  RightPortType=p1  LConnTagsString=__newl0|__newl1|__newl2|__newl3|__newl4|__newl5|__newl6|__newl7|__newl8|__newl9  RConnTagsString=__newr0|__newr1|__newr2  mask(Bus){in=10, out=3, p2q=230, p3_4q=[1.00  0.00], p5q=3, p6q=1}
      mask prompts: in "Number of inputs:"; out "Number of outputs:"; p2q "Voltage Rating [kV]"; p3_4q "Voltage initial guess [p.u.  rad]"; p5q "Area number"; p6q "Region number"
      mask help: Bus block.
      mask init:
      | fm_inout
      mask CallbackString: ||||fm_block|
      mask Display: plot([0 1 1 0 0],[0 0 1 1 0])
  Bus116 : PMComponent  Tag=PSATblock  Description=Connection  Orientation=down  PhysicalDomain=psatdomain  LeftPortType=p1  RightPortType=p1  LConnTagsString=__newl0|__newl1|__newl2|__newl3  RConnTagsString=__newr0|__newr1|__newr2|__newr3  mask(Bus){in=4, out=4, p2q=230, p3_4q=[1.00  0.00], p5q=3, p6q=1}
      mask prompts: in "Number of inputs:"; out "Number of outputs:"; p2q "Voltage Rating [kV]"; p3_4q "Voltage initial guess [p.u.  rad]"; p5q "Area number"; p6q "Region number"
      mask help: Bus block.
      mask init:
      | fm_inout
      mask CallbackString: ||||fm_block|
      mask Display: plot([0 1 1 0 0],[0 0 1 1 0])
  Bus117 : PMComponent  Tag=PSATblock  Description=Connection  Orientation=left  PhysicalDomain=psatdomain  LeftPortType=p1  RightPortType=p1  LConnTagsString=__newl0|__newl1  RConnTagsString=__newr0  mask(Bus){in=2, out=1, p2q=230, p3_4q=[1.00   0.00], p5q=3, p6q=1}
      mask prompts: in "Number of inputs:"; out "Number of outputs:"; p2q "Voltage Rating [kV]"; p3_4q "Voltage initial guess [p.u.  rad]"; p5q "Area number"; p6q "Region number"
      mask help: Bus block.
      mask init:
      | fm_inout
      mask CallbackString: ||||fm_block|
      mask Display: plot([0 1 1 0 0],[0 0 1 1 0])
  Bus118 : PMComponent  Tag=PSATblock  Description=Connection  Orientation=down  PhysicalDomain=psatdomain  LeftPortType=p1  RightPortType=p1  LConnTagsString=__newl0|__newl1  RConnTagsString=__newr0|__newr1|__newr2|__newr3|__newr4  mask(Bus){in=2, out=5, p2q=230, p3_4q=[1.00  0.00], p5q=3, p6q=1}
      mask prompts: in "Number of inputs:"; out "Number of outputs:"; p2q "Voltage Rating [kV]"; p3_4q "Voltage initial guess [p.u.  rad]"; p5q "Area number"; p6q "Region number"
      mask help: Bus block.
      mask init:
      | fm_inout
      mask CallbackString: ||||fm_block|
      mask Display: plot([0 1 1 0 0],[0 0 1 1 0])
  Bus119 : PMComponent  Tag=PSATblock  Description=Connection  Orientation=up  PhysicalDomain=psatdomain  LeftPortType=p1  RightPortType=p1  RConnTagsString=__newr0|__newr1|__newr2|__newr3|__newr4  mask(Bus){in=0, out=5, p2q=230, p3_4q=[1.00  0.00], p5q=3, p6q=1}
      mask prompts: in "Number of inputs:"; out "Number of outputs:"; p2q "Voltage Rating [kV]"; p3_4q "Voltage initial guess [p.u.  rad]"; p5q "Area number"; p6q "Region number"
      mask help: Bus block.
      mask init:
      | fm_inout
      mask CallbackString: ||||fm_block|
      mask Display: plot([0 1 1 0 0],[0 0 1 1 0])
  Bus120 : PMComponent  Tag=PSATblock  Description=Connection  Orientation=down  PhysicalDomain=psatdomain  LeftPortType=p1  RightPortType=p1  LConnTagsString=__newl0|__newl1|__newl2|__newl3  RConnTagsString=__newr0|__newr1  mask(Bus){in=4, out=2, p2q=230, p3_4q=[1.00  0.00], p5q=3, p6q=1}
      mask prompts: in "Number of inputs:"; out "Number of outputs:"; p2q "Voltage Rating [kV]"; p3_4q "Voltage initial guess [p.u.  rad]"; p5q "Area number"; p6q "Region number"
      mask help: Bus block.
      mask init:
      | fm_inout
      mask CallbackString: ||||fm_block|
      mask Display: plot([0 1 1 0 0],[0 0 1 1 0])
  Bus121 : PMComponent  Tag=PSATblock  Description=Connection  Orientation=down  PhysicalDomain=psatdomain  LeftPortType=p1  RightPortType=p1  LConnTagsString=__newl0|__newl1|__newl2|__newl3  RConnTagsString=__newr0|__newr1|__newr2  mask(Bus){in=4, out=3, p2q=230, p3_4q=[1.00  0.00], p5q=3, p6q=1}
      mask prompts: in "Number of inputs:"; out "Number of outputs:"; p2q "Voltage Rating [kV]"; p3_4q "Voltage initial guess [p.u.  rad]"; p5q "Area number"; p6q "Region number"
      mask help: Bus block.
      mask init:
      | fm_inout
      mask CallbackString: ||||fm_block|
      mask Display: plot([0 1 1 0 0],[0 0 1 1 0])
  Bus122 : PMComponent  Tag=PSATblock  Description=Connection  Orientation=down  PhysicalDomain=psatdomain  LeftPortType=p1  RightPortType=p1  LConnTagsString=__newl0|__newl1|__newl2|__newl3|__newl4|__newl5|__newl6|__newl7  RConnTagsString=__newr0  mask(Bus){in=8, out=1, p2q=230, p3_4q=[1.00  0.00], p5q=3, p6q=1}
      mask prompts: in "Number of inputs:"; out "Number of outputs:"; p2q "Voltage Rating [kV]"; p3_4q "Voltage initial guess [p.u.  rad]"; p5q "Area number"; p6q "Region number"
      mask help: Bus block.
      mask init:
      | fm_inout
      mask CallbackString: ||||fm_block|
      mask Display: plot([0 1 1 0 0],[0 0 1 1 0])
  Bus123 : PMComponent  Tag=PSATblock  Description=Connection  Orientation=left  PhysicalDomain=psatdomain  LeftPortType=p1  RightPortType=p1  LConnTagsString=__newl0|__newl1|__newl2|__newl3|__newl4  RConnTagsString=__newr0|__newr1|__newr2  mask(Bus){in=5, out=3, p2q=230, p3_4q=[1.00   0.00], p5q=3, p6q=1}
      mask prompts: in "Number of inputs:"; out "Number of outputs:"; p2q "Voltage Rating [kV]"; p3_4q "Voltage initial guess [p.u.  rad]"; p5q "Area number"; p6q "Region number"
      mask help: Bus block.
      mask init:
      | fm_inout
      mask CallbackString: ||||fm_block|
      mask Display: plot([0 1 1 0 0],[0 0 1 1 0])
  Bus124 : PMComponent  Tag=PSATblock  Description=Connection  Orientation=down  PhysicalDomain=psatdomain  LeftPortType=p1  RightPortType=p1  LConnTagsString=__newl0  RConnTagsString=__newr0  mask(Bus){in=1, out=1, p2q=230, p3_4q=[1.00  0.00], p5q=3, p6q=1}
      mask prompts: in "Number of inputs:"; out "Number of outputs:"; p2q "Voltage Rating [kV]"; p3_4q "Voltage initial guess [p.u.  rad]"; p5q "Area number"; p6q "Region number"
      mask help: Bus block.
      mask init:
      | fm_inout
      mask CallbackString: ||||fm_block|
      mask Display: plot([0 1 1 0 0],[0 0 1 1 0])
  Dem101 : PMComponent  Tag=PSATblock  Description=OPF & CPF  Orientation=up  PhysicalDomain=psatdomain  LeftPortType=p1  RightPortType=p1  LConnTagsString=__newl0  mask(Demand){p2q=100, p3q=1.188, p4q=0.242, p5_6q=[1.188*1.2  1.188*0.8], p8_9_10q=[0.00  18  0.00], p11_12_13q=[0.00  0.00  0.00], p14q=off, p15q=0, p16_17q=[0 0], out=0, p18q=on}
      mask prompts: p2q "Power Rating [MVA]"; p3q "Active Power [p.u.]"; p4q "Reactive Power [p.u.]"; p5_6q "Max and Min Power Demand [p.u.  p.u.]"; p8_9_10q "Cost = a + b*P + c*P^2 [$/h, $/MWh, $/(MW)^2 h]"; p11_12_13q "Cost = a + b*Q + c*Q^2 [$/h, $/MVArh, $/(MVAr)^2 h]"; p14q "Allow Unit Commitment"; p15q "Tie Breaking Cost [$/h]"; p16_17q "Up and down congestion costs [$/h $/h]"; out "Number of Output Signals"; p18q "Connected"
      mask help: This block defines a constant power load for bifurcation and market studies.
      mask init:
      | fm_inout;
      | [xs,ys]=fm_draw('$');
      mask StyleString: edit,edit,edit,edit,edit,edit,checkbox,edit,edit,popup(0|1),checkbox
      mask CallbackString: ||||||||||fm_block
      mask Display:
      | plot([ 1.0000    -0.5   -0.5  1],[ 0    0.866    -0.866    0])
      | color('blue')
      | plot(0.6*xs,0.6*ys)
  Dem102 : PMComponent  Tag=PSATblock  Description=OPF & CPF  Orientation=up  PhysicalDomain=psatdomain  LeftPortType=p1  RightPortType=p1  LConnTagsString=__newl0  mask(Demand){p2q=100, p3q=1.067, p4q=0.22, p5_6q=[1.067*1.2  1.067*0.8], p8_9_10q=[0.00  25  0.00], p11_12_13q=[0.00  0.00  0.00], p14q=off, p15q=0, p16_17q=[0 0], out=0, p18q=on}
      mask prompts: p2q "Power Rating [MVA]"; p3q "Active Power [p.u.]"; p4q "Reactive Power [p.u.]"; p5_6q "Max and Min Power Demand [p.u.  p.u.]"; p8_9_10q "Cost = a + b*P + c*P^2 [$/h, $/MWh, $/(MW)^2 h]"; p11_12_13q "Cost = a + b*Q + c*Q^2 [$/h, $/MVArh, $/(MVAr)^2 h]"; p14q "Allow Unit Commitment"; p15q "Tie Breaking Cost [$/h]"; p16_17q "Up and down congestion costs [$/h $/h]"; out "Number of Output Signals"; p18q "Connected"
      mask help: This block defines a constant power load for bifurcation and market studies.
      mask init:
      | fm_inout;
      | [xs,ys]=fm_draw('$');
      mask StyleString: edit,edit,edit,edit,edit,edit,checkbox,edit,edit,popup(0|1),checkbox
      mask CallbackString: ||||||||||fm_block
      mask Display:
      | plot([ 1.0000    -0.5   -0.5  1],[ 0    0.866    -0.866    0])
      | color('blue')
      | plot(0.6*xs,0.6*ys)
  Dem103 : PMComponent  Tag=PSATblock  Description=OPF & CPF  Orientation=left  PhysicalDomain=psatdomain  LeftPortType=p1  RightPortType=p1  LConnTagsString=__newl0  mask(Demand){p2q=100, p3q=1.98, p4q=0.407, p5_6q=[1.98*1.2  1.98*0.8], p8_9_10q=[0.00  19  0.00], p11_12_13q=[0.00  0.00  0.00], p14q=off, p15q=0, p16_17q=[0 0], out=0, p18q=on}
      mask prompts: p2q "Power Rating [MVA]"; p3q "Active Power [p.u.]"; p4q "Reactive Power [p.u.]"; p5_6q "Max and Min Power Demand [p.u.  p.u.]"; p8_9_10q "Cost = a + b*P + c*P^2 [$/h, $/MWh, $/(MW)^2 h]"; p11_12_13q "Cost = a + b*Q + c*Q^2 [$/h, $/MVArh, $/(MVAr)^2 h]"; p14q "Allow Unit Commitment"; p15q "Tie Breaking Cost [$/h]"; p16_17q "Up and down congestion costs [$/h $/h]"; out "Number of Output Signals"; p18q "Connected"
      mask help: This block defines a constant power load for bifurcation and market studies.
      mask init:
      | fm_inout;
      | [xs,ys]=fm_draw('$');
      mask StyleString: edit,edit,edit,edit,edit,edit,checkbox,edit,edit,popup(0|1),checkbox
      mask CallbackString: ||||||||||fm_block
      mask Display:
      | plot([ 1.0000    -0.5   -0.5  1],[ 0    0.866    -0.866    0])
      | color('blue')
      | plot(0.6*xs,0.6*ys)
  Dem104 : PMComponent  Tag=PSATblock  Description=OPF & CPF  Orientation=left  PhysicalDomain=psatdomain  LeftPortType=p1  RightPortType=p1  LConnTagsString=__newl0  mask(Demand){p2q=100, p3q=0.814, p4q=0.165, p5_6q=[0.814*1.2  0.814*0.8], p8_9_10q=[0.00  24  0.00], p11_12_13q=[0.00  0.00  0.00], p14q=off, p15q=0, p16_17q=[0 0], out=0, p18q=on}
      mask prompts: p2q "Power Rating [MVA]"; p3q "Active Power [p.u.]"; p4q "Reactive Power [p.u.]"; p5_6q "Max and Min Power Demand [p.u.  p.u.]"; p8_9_10q "Cost = a + b*P + c*P^2 [$/h, $/MWh, $/(MW)^2 h]"; p11_12_13q "Cost = a + b*Q + c*Q^2 [$/h, $/MVArh, $/(MVAr)^2 h]"; p14q "Allow Unit Commitment"; p15q "Tie Breaking Cost [$/h]"; p16_17q "Up and down congestion costs [$/h $/h]"; out "Number of Output Signals"; p18q "Connected"
      mask help: This block defines a constant power load for bifurcation and market studies.
      mask init:
      | fm_inout;
      | [xs,ys]=fm_draw('$');
      mask StyleString: edit,edit,edit,edit,edit,edit,checkbox,edit,edit,popup(0|1),checkbox
      mask CallbackString: ||||||||||fm_block
      mask Display:
      | plot([ 1.0000    -0.5   -0.5  1],[ 0    0.866    -0.866    0])
      | color('blue')
      | plot(0.6*xs,0.6*ys)
  Dem105 : PMComponent  Tag=PSATblock  Description=OPF & CPF  Orientation=down  PhysicalDomain=psatdomain  LeftPortType=p1  RightPortType=p1  LConnTagsString=__newl0  mask(Demand){p2q=100, p3q=0.781, p4q=0.154, p5_6q=[0.781*1.2 0.781*0.8], p8_9_10q=[0.00  22  0.00], p11_12_13q=[0.00  0.00  0.00], p14q=off, p15q=0, p16_17q=[0 0], out=0, p18q=on}
      mask prompts: p2q "Power Rating [MVA]"; p3q "Active Power [p.u.]"; p4q "Reactive Power [p.u.]"; p5_6q "Max and Min Power Demand [p.u.  p.u.]"; p8_9_10q "Cost = a + b*P + c*P^2 [$/h, $/MWh, $/(MW)^2 h]"; p11_12_13q "Cost = a + b*Q + c*Q^2 [$/h, $/MVArh, $/(MVAr)^2 h]"; p14q "Allow Unit Commitment"; p15q "Tie Breaking Cost [$/h]"; p16_17q "Up and down congestion costs [$/h $/h]"; out "Number of Output Signals"; p18q "Connected"
      mask help: This block defines a constant power load for bifurcation and market studies.
      mask init:
      | fm_inout;
      | [xs,ys]=fm_draw('$');
      mask StyleString: edit,edit,edit,edit,edit,edit,checkbox,edit,edit,popup(0|1),checkbox
      mask CallbackString: ||||||||||fm_block
      mask Display:
      | plot([ 1.0000    -0.5   -0.5  1],[ 0    0.866    -0.866    0])
      | color('blue')
      | plot(0.6*xs,0.6*ys)
  Dem106 : PMComponent  Tag=PSATblock  Description=OPF & CPF  PhysicalDomain=psatdomain  LeftPortType=p1  RightPortType=p1  LConnTagsString=__newl0  mask(Demand){p2q=100, p3q=1.496, p4q=0.308, p5_6q=[1.496*1.2  1.496*0.8], p8_9_10q=[0.00  19  0.00], p11_12_13q=[0.00  0.00  0.00], p14q=off, p15q=0, p16_17q=[0 0], out=0, p18q=on}
      mask prompts: p2q "Power Rating [MVA]"; p3q "Active Power [p.u.]"; p4q "Reactive Power [p.u.]"; p5_6q "Max and Min Power Demand [p.u.  p.u.]"; p8_9_10q "Cost = a + b*P + c*P^2 [$/h, $/MWh, $/(MW)^2 h]"; p11_12_13q "Cost = a + b*Q + c*Q^2 [$/h, $/MVArh, $/(MVAr)^2 h]"; p14q "Allow Unit Commitment"; p15q "Tie Breaking Cost [$/h]"; p16_17q "Up and down congestion costs [$/h $/h]"; out "Number of Output Signals"; p18q "Connected"
      mask help: This block defines a constant power load for bifurcation and market studies.
      mask init:
      | fm_inout;
      | [xs,ys]=fm_draw('$');
      mask StyleString: edit,edit,edit,edit,edit,edit,checkbox,edit,edit,popup(0|1),checkbox
      mask CallbackString: ||||||||||fm_block
      mask Display:
      | plot([ 1.0000    -0.5   -0.5  1],[ 0    0.866    -0.866    0])
      | color('blue')
      | plot(0.6*xs,0.6*ys)
  Dem107 : PMComponent  Tag=PSATblock  Description=OPF & CPF  Orientation=up  PhysicalDomain=psatdomain  LeftPortType=p1  RightPortType=p1  LConnTagsString=__newl0  mask(Demand){p2q=100, p3q=1.375, p4q=0.275, p5_6q=[1.375*1.2  1.375*0.8], p8_9_10q=[0.00  22  0.00], p11_12_13q=[0.00  0.00  0.00], p14q=off, p15q=0, p16_17q=[0 0], out=0, p18q=on}
      mask prompts: p2q "Power Rating [MVA]"; p3q "Active Power [p.u.]"; p4q "Reactive Power [p.u.]"; p5_6q "Max and Min Power Demand [p.u.  p.u.]"; p8_9_10q "Cost = a + b*P + c*P^2 [$/h, $/MWh, $/(MW)^2 h]"; p11_12_13q "Cost = a + b*Q + c*Q^2 [$/h, $/MVArh, $/(MVAr)^2 h]"; p14q "Allow Unit Commitment"; p15q "Tie Breaking Cost [$/h]"; p16_17q "Up and down congestion costs [$/h $/h]"; out "Number of Output Signals"; p18q "Connected"
      mask help: This block defines a constant power load for bifurcation and market studies.
      mask init:
      | fm_inout;
      | [xs,ys]=fm_draw('$');
      mask StyleString: edit,edit,edit,edit,edit,edit,checkbox,edit,edit,popup(0|1),checkbox
      mask CallbackString: ||||||||||fm_block
      mask Display:
      | plot([ 1.0000    -0.5   -0.5  1],[ 0    0.866    -0.866    0])
      | color('blue')
      | plot(0.6*xs,0.6*ys)
  Dem108 : PMComponent  Tag=PSATblock  Description=OPF & CPF  PhysicalDomain=psatdomain  LeftPortType=p1  RightPortType=p1  LConnTagsString=__newl0  mask(Demand){p2q=100, p3q=1.881, p4q=0.385, p5_6q=[1.881*1.2  1.881*0.8], p8_9_10q=[0.00  20  0.00], p11_12_13q=[0.00  0.00  0.00], p14q=off, p15q=0, p16_17q=[0 0], out=0, p18q=on}
      mask prompts: p2q "Power Rating [MVA]"; p3q "Active Power [p.u.]"; p4q "Reactive Power [p.u.]"; p5_6q "Max and Min Power Demand [p.u.  p.u.]"; p8_9_10q "Cost = a + b*P + c*P^2 [$/h, $/MWh, $/(MW)^2 h]"; p11_12_13q "Cost = a + b*Q + c*Q^2 [$/h, $/MVArh, $/(MVAr)^2 h]"; p14q "Allow Unit Commitment"; p15q "Tie Breaking Cost [$/h]"; p16_17q "Up and down congestion costs [$/h $/h]"; out "Number of Output Signals"; p18q "Connected"
      mask help: This block defines a constant power load for bifurcation and market studies.
      mask init:
      | fm_inout;
      | [xs,ys]=fm_draw('$');
      mask StyleString: edit,edit,edit,edit,edit,edit,checkbox,edit,edit,popup(0|1),checkbox
      mask CallbackString: ||||||||||fm_block
      mask Display:
      | plot([ 1.0000    -0.5   -0.5  1],[ 0    0.866    -0.866    0])
      | color('blue')
      | plot(0.6*xs,0.6*ys)
  Dem109 : PMComponent  Tag=PSATblock  Description=OPF & CPF  Orientation=down  PhysicalDomain=psatdomain  LeftPortType=p1  RightPortType=p1  LConnTagsString=__newl0  mask(Demand){p2q=100, p3q=1.925, p4q=0.396, p5_6q=[1.925*1.2  1.925*0.8], p8_9_10q=[0.00  20  0.00], p11_12_13q=[0.00  0.00  0.00], p14q=off, p15q=0, p16_17q=[0 0], out=0, p18q=on}
      mask prompts: p2q "Power Rating [MVA]"; p3q "Active Power [p.u.]"; p4q "Reactive Power [p.u.]"; p5_6q "Max and Min Power Demand [p.u.  p.u.]"; p8_9_10q "Cost = a + b*P + c*P^2 [$/h, $/MWh, $/(MW)^2 h]"; p11_12_13q "Cost = a + b*Q + c*Q^2 [$/h, $/MVArh, $/(MVAr)^2 h]"; p14q "Allow Unit Commitment"; p15q "Tie Breaking Cost [$/h]"; p16_17q "Up and down congestion costs [$/h $/h]"; out "Number of Output Signals"; p18q "Connected"
      mask help: This block defines a constant power load for bifurcation and market studies.
      mask init:
      | fm_inout;
      | [xs,ys]=fm_draw('$');
      mask StyleString: edit,edit,edit,edit,edit,edit,checkbox,edit,edit,popup(0|1),checkbox
      mask CallbackString: ||||||||||fm_block
      mask Display:
      | plot([ 1.0000    -0.5   -0.5  1],[ 0    0.866    -0.866    0])
      | color('blue')
      | plot(0.6*xs,0.6*ys)
  Dem110 : PMComponent  Tag=PSATblock  Description=OPF & CPF  Orientation=down  PhysicalDomain=psatdomain  LeftPortType=p1  RightPortType=p1  LConnTagsString=__newl0  mask(Demand){p2q=100, p3q=2.145, p4q=0.44, p5_6q=[2.145*1.2  2.145*0.8], p8_9_10q=[0.00  19  0.00], p11_12_13q=[0.00  0.00  0.00], p14q=off, p15q=0, p16_17q=[0 0], out=0, p18q=on}
      mask prompts: p2q "Power Rating [MVA]"; p3q "Active Power [p.u.]"; p4q "Reactive Power [p.u.]"; p5_6q "Max and Min Power Demand [p.u.  p.u.]"; p8_9_10q "Cost = a + b*P + c*P^2 [$/h, $/MWh, $/(MW)^2 h]"; p11_12_13q "Cost = a + b*Q + c*Q^2 [$/h, $/MVArh, $/(MVAr)^2 h]"; p14q "Allow Unit Commitment"; p15q "Tie Breaking Cost [$/h]"; p16_17q "Up and down congestion costs [$/h $/h]"; out "Number of Output Signals"; p18q "Connected"
      mask help: This block defines a constant power load for bifurcation and market studies.
      mask init:
      | fm_inout;
      | [xs,ys]=fm_draw('$');
      mask StyleString: edit,edit,edit,edit,edit,edit,checkbox,edit,edit,popup(0|1),checkbox
      mask CallbackString: ||||||||||fm_block
      mask Display:
      | plot([ 1.0000    -0.5   -0.5  1],[ 0    0.866    -0.866    0])
      | color('blue')
      | plot(0.6*xs,0.6*ys)
  Dem113 : PMComponent  Tag=PSATblock  Description=OPF & CPF  Orientation=left  PhysicalDomain=psatdomain  LeftPortType=p1  RightPortType=p1  LConnTagsString=__newl0  mask(Demand){p2q=100, p3q=2.915, p4q=0.594, p5_6q=[2.915*1.2 2.915*0.8], p8_9_10q=[0.00  19  0.00], p11_12_13q=[0.00  0.00  0.00], p14q=off, p15q=0, p16_17q=[0 0], out=0, p18q=on}
      mask prompts: p2q "Power Rating [MVA]"; p3q "Active Power [p.u.]"; p4q "Reactive Power [p.u.]"; p5_6q "Max and Min Power Demand [p.u.  p.u.]"; p8_9_10q "Cost = a + b*P + c*P^2 [$/h, $/MWh, $/(MW)^2 h]"; p11_12_13q "Cost = a + b*Q + c*Q^2 [$/h, $/MVArh, $/(MVAr)^2 h]"; p14q "Allow Unit Commitment"; p15q "Tie Breaking Cost [$/h]"; p16_17q "Up and down congestion costs [$/h $/h]"; out "Number of Output Signals"; p18q "Connected"
      mask help: This block defines a constant power load for bifurcation and market studies.
      mask init:
      | fm_inout;
      | [xs,ys]=fm_draw('$');
      mask StyleString: edit,edit,edit,edit,edit,edit,checkbox,edit,edit,popup(0|1),checkbox
      mask CallbackString: ||||||||||fm_block
      mask Display:
      | plot([ 1.0000    -0.5   -0.5  1],[ 0    0.866    -0.866    0])
      | color('blue')
      | plot(0.6*xs,0.6*ys)
  Dem114 : PMComponent  Tag=PSATblock  Description=OPF & CPF  PhysicalDomain=psatdomain  LeftPortType=p1  RightPortType=p1  LConnTagsString=__newl0  mask(Demand){p2q=100, p3q=2.134, p4q=0.429, p5_6q=[2.134*1.2  2.134*0.8], p8_9_10q=[0.00  25  0.00], p11_12_13q=[0.00  0.00  0.00], p14q=off, p15q=0, p16_17q=[0 0], out=0, p18q=on}
      mask prompts: p2q "Power Rating [MVA]"; p3q "Active Power [p.u.]"; p4q "Reactive Power [p.u.]"; p5_6q "Max and Min Power Demand [p.u.  p.u.]"; p8_9_10q "Cost = a + b*P + c*P^2 [$/h, $/MWh, $/(MW)^2 h]"; p11_12_13q "Cost = a + b*Q + c*Q^2 [$/h, $/MVArh, $/(MVAr)^2 h]"; p14q "Allow Unit Commitment"; p15q "Tie Breaking Cost [$/h]"; p16_17q "Up and down congestion costs [$/h $/h]"; out "Number of Output Signals"; p18q "Connected"
      mask help: This block defines a constant power load for bifurcation and market studies.
      mask init:
      | fm_inout;
      | [xs,ys]=fm_draw('$');
      mask StyleString: edit,edit,edit,edit,edit,edit,checkbox,edit,edit,popup(0|1),checkbox
      mask CallbackString: ||||||||||fm_block
      mask Display:
      | plot([ 1.0000    -0.5   -0.5  1],[ 0    0.866    -0.866    0])
      | color('blue')
      | plot(0.6*xs,0.6*ys)
  Dem115 : PMComponent  Tag=PSATblock  Description=OPF & CPF  Orientation=down  PhysicalDomain=psatdomain  LeftPortType=p1  RightPortType=p1  LConnTagsString=__newl0  mask(Demand){p2q=100, p3q=3.847, p4q=0.704, p5_6q=[3.847*1.2  3.847*0.8], p8_9_10q=[0.00  25  0.00], p11_12_13q=[0.00  0.00  0.00], p14q=off, p15q=0, p16_17q=[0 0], out=0, p18q=on}
      mask prompts: p2q "Power Rating [MVA]"; p3q "Active Power [p.u.]"; p4q "Reactive Power [p.u.]"; p5_6q "Max and Min Power Demand [p.u.  p.u.]"; p8_9_10q "Cost = a + b*P + c*P^2 [$/h, $/MWh, $/(MW)^2 h]"; p11_12_13q "Cost = a + b*Q + c*Q^2 [$/h, $/MVArh, $/(MVAr)^2 h]"; p14q "Allow Unit Commitment"; p15q "Tie Breaking Cost [$/h]"; p16_17q "Up and down congestion costs [$/h $/h]"; out "Number of Output Signals"; p18q "Connected"
      mask help: This block defines a constant power load for bifurcation and market studies.
      mask init:
      | fm_inout;
      | [xs,ys]=fm_draw('$');
      mask StyleString: edit,edit,edit,edit,edit,edit,checkbox,edit,edit,popup(0|1),checkbox
      mask CallbackString: ||||||||||fm_block
      mask Display:
      | plot([ 1.0000    -0.5   -0.5  1],[ 0    0.866    -0.866    0])
      | color('blue')
      | plot(0.6*xs,0.6*ys)
  Dem116 : PMComponent  Tag=PSATblock  Description=OPF & CPF  Orientation=down  PhysicalDomain=psatdomain  LeftPortType=p1  RightPortType=p1  LConnTagsString=__newl0  mask(Demand){p2q=100, p3q=1.1, p4q=0.22, p5_6q=[1.1*1.2  1.1*0.8], p8_9_10q=[0.00  23  0.00], p11_12_13q=[0.00  0.00  0.00], p14q=off, p15q=0, p16_17q=[0 0], out=0, p18q=on}
      mask prompts: p2q "Power Rating [MVA]"; p3q "Active Power [p.u.]"; p4q "Reactive Power [p.u.]"; p5_6q "Max and Min Power Demand [p.u.  p.u.]"; p8_9_10q "Cost = a + b*P + c*P^2 [$/h, $/MWh, $/(MW)^2 h]"; p11_12_13q "Cost = a + b*Q + c*Q^2 [$/h, $/MVArh, $/(MVAr)^2 h]"; p14q "Allow Unit Commitment"; p15q "Tie Breaking Cost [$/h]"; p16_17q "Up and down congestion costs [$/h $/h]"; out "Number of Output Signals"; p18q "Connected"
      mask help: This block defines a constant power load for bifurcation and market studies.
      mask init:
      | fm_inout;
      | [xs,ys]=fm_draw('$');
      mask StyleString: edit,edit,edit,edit,edit,edit,checkbox,edit,edit,popup(0|1),checkbox
      mask CallbackString: ||||||||||fm_block
      mask Display:
      | plot([ 1.0000    -0.5   -0.5  1],[ 0    0.866    -0.866    0])
      | color('blue')
      | plot(0.6*xs,0.6*ys)
  Dem118 : PMComponent  Tag=PSATblock  Description=OPF & CPF  Orientation=left  PhysicalDomain=psatdomain  LeftPortType=p1  RightPortType=p1  LConnTagsString=__newl0  mask(Demand){p2q=100, p3q=3.663, p4q=0.748, p5_6q=[3.663*1.2  3.663*0.8], p8_9_10q=[0.00  18  0.00], p11_12_13q=[0.00  0.00  0.00], p14q=off, p15q=0, p16_17q=[0 0], out=0, p18q=on}
      mask prompts: p2q "Power Rating [MVA]"; p3q "Active Power [p.u.]"; p4q "Reactive Power [p.u.]"; p5_6q "Max and Min Power Demand [p.u.  p.u.]"; p8_9_10q "Cost = a + b*P + c*P^2 [$/h, $/MWh, $/(MW)^2 h]"; p11_12_13q "Cost = a + b*Q + c*Q^2 [$/h, $/MVArh, $/(MVAr)^2 h]"; p14q "Allow Unit Commitment"; p15q "Tie Breaking Cost [$/h]"; p16_17q "Up and down congestion costs [$/h $/h]"; out "Number of Output Signals"; p18q "Connected"
      mask help: This block defines a constant power load for bifurcation and market studies.
      mask init:
      | fm_inout;
      | [xs,ys]=fm_draw('$');
      mask StyleString: edit,edit,edit,edit,edit,edit,checkbox,edit,edit,popup(0|1),checkbox
      mask CallbackString: ||||||||||fm_block
      mask Display:
      | plot([ 1.0000    -0.5   -0.5  1],[ 0    0.866    -0.866    0])
      | color('blue')
      | plot(0.6*xs,0.6*ys)
  Dem119 : PMComponent  Tag=PSATblock  Description=OPF & CPF  Orientation=up  PhysicalDomain=psatdomain  LeftPortType=p1  RightPortType=p1  LConnTagsString=__newl0  mask(Demand){p2q=100, p3q=1.991, p4q=0.407, p5_6q=[1.991*1.2  1.991*0.8], p8_9_10q=[0.00  19  0.00], p11_12_13q=[0.00  0.00  0.00], p14q=off, p15q=0, p16_17q=[0 0], out=0, p18q=on}
      mask prompts: p2q "Power Rating [MVA]"; p3q "Active Power [p.u.]"; p4q "Reactive Power [p.u.]"; p5_6q "Max and Min Power Demand [p.u.  p.u.]"; p8_9_10q "Cost = a + b*P + c*P^2 [$/h, $/MWh, $/(MW)^2 h]"; p11_12_13q "Cost = a + b*Q + c*Q^2 [$/h, $/MVArh, $/(MVAr)^2 h]"; p14q "Allow Unit Commitment"; p15q "Tie Breaking Cost [$/h]"; p16_17q "Up and down congestion costs [$/h $/h]"; out "Number of Output Signals"; p18q "Connected"
      mask help: This block defines a constant power load for bifurcation and market studies.
      mask init:
      | fm_inout;
      | [xs,ys]=fm_draw('$');
      mask StyleString: edit,edit,edit,edit,edit,edit,checkbox,edit,edit,popup(0|1),checkbox
      mask CallbackString: ||||||||||fm_block
      mask Display:
      | plot([ 1.0000    -0.5   -0.5  1],[ 0    0.866    -0.866    0])
      | color('blue')
      | plot(0.6*xs,0.6*ys)
  Dem120 : PMComponent  Tag=PSATblock  Description=OPF & CPF  Orientation=down  PhysicalDomain=psatdomain  LeftPortType=p1  RightPortType=p1  LConnTagsString=__newl0  mask(Demand){p2q=100, p3q=1.408, p4q=0.286, p5_6q=[1.408*1.2  1.408*0.8], p8_9_10q=[0.00  23  0.00], p11_12_13q=[0.00  0.00 0.00], p14q=off, p15q=0, p16_17q=[0 0], out=0, p18q=on}
      mask prompts: p2q "Power Rating [MVA]"; p3q "Active Power [p.u.]"; p4q "Reactive Power [p.u.]"; p5_6q "Max and Min Power Demand [p.u.  p.u.]"; p8_9_10q "Cost = a + b*P + c*P^2 [$/h, $/MWh, $/(MW)^2 h]"; p11_12_13q "Cost = a + b*Q + c*Q^2 [$/h, $/MVArh, $/(MVAr)^2 h]"; p14q "Allow Unit Commitment"; p15q "Tie Breaking Cost [$/h]"; p16_17q "Up and down congestion costs [$/h $/h]"; out "Number of Output Signals"; p18q "Connected"
      mask help: This block defines a constant power load for bifurcation and market studies.
      mask init:
      | fm_inout;
      | [xs,ys]=fm_draw('$');
      mask StyleString: edit,edit,edit,edit,edit,edit,checkbox,edit,edit,popup(0|1),checkbox
      mask CallbackString: ||||||||||fm_block
      mask Display:
      | plot([ 1.0000    -0.5   -0.5  1],[ 0    0.866    -0.866    0])
      | color('blue')
      | plot(0.6*xs,0.6*ys)
  Gen101 : PMComponent  Tag=PSATblock  Description=Power Flow  Orientation=up  PhysicalDomain=psatdomain  LeftPortType=p1  RightPortType=p1  RConnTagsString=__newr0  mask(PV){p2_3q=[100  138], p4q=1.72, p5q=1.035, p6_7q=[0.8  -0.5], p8_9q=[1.05  0.95], p10q=1, p11q=on}
      mask prompts: p2_3q "Power and Voltage Ratings [MVA, kV]"; p4q "Active Power [p.u.]"; p5q "Voltage Magnitude [p.u.]"; p6_7q "Qmax and Qmin [p.u.  p.u.]"; p8_9q "Vmax and Vmin [p.u.  p.u.]"; p10q "Loss Participation Factor"; p11q "Connected"
      mask help:
      | This block defines a PV bus for load flow studies:
      |
      | P = Pcost.
      | V = Vdes.
      mask init:
      | [x,y] = fm_draw('circle');
      | [xp,yp] = fm_draw('P');
      mask CallbackString: ||||||fm_block
      mask Display:
      | plot(x,y)
      | color('blue')
      | plot(0.3*xp-0.35,0.6*yp,[0.1 0.3 0.5],[0.3 -0.3 0.3])
  Gen102 : PMComponent  Tag=PSATblock  Description=Power Flow  Orientation=up  PhysicalDomain=psatdomain  LeftPortType=p1  RightPortType=p1  RConnTagsString=__newr0  mask(PV){p2_3q=[100  138], p4q=1.72, p5q=1.035, p6_7q=[0.8  -0.5], p8_9q=[1.05  0.95], p10q=1, p11q=on}
      mask prompts: p2_3q "Power and Voltage Ratings [MVA, kV]"; p4q "Active Power [p.u.]"; p5q "Voltage Magnitude [p.u.]"; p6_7q "Qmax & Qmin [p.u.  p.u.]"; p8_9q "Vmax & Vmin [p.u.  p.u.]"; p10q "Loss Participation Factor"; p11q "Connected"
      mask help:
      | This block defines a PV bus for load flow studies:
      |
      | P = Pcost.
      | V = Vdes.
      mask init:
      | [x,y] = fm_draw('circle');
      | [xp,yp] = fm_draw('P');
      mask CallbackString: ||||||fm_block
      mask Display:
      | plot(x,y)
      | color('blue')
      | plot(0.3*xp-0.35,0.6*yp,[0.1 0.3 0.5],[0.3 -0.3 0.3])
  Gen107 : fm_lib/Power Flow/PV  Tag=PSATblock  Description=Power Flow  Orientation=up  PhysicalDomain=psatdomain  SubClassName=unknown  LeftPortType=p1  RightPortType=p1  RConnTagsString=__newr0  p2_3q="[100  138]"  p4q=2.40  p5q=1.025  p6_7q="[1.8  0.0]"  p8_9q="[1.05  0.95]"  p10q=1  p11q=on
  Gen113 : fm_lib/Power Flow/Slack  Tag=PSATblock  Description=Power Flow  Orientation=left  PhysicalDomain=psatdomain  SubClassName=unknown  LeftPortType=p1  RightPortType=p1  RConnTagsString=__newr0  p2_3q="[100  230]"  p4q=1.02  p5q=0.00  p6_7q="[2.4  0]"  p8_9q="[1.05  0.95]"  p10q=4.7321  p11q=1  p12q=on  p13q=on
  Gen114 : PMComponent  Tag=PSATblock  Description=Power Flow  PhysicalDomain=psatdomain  LeftPortType=p1  RightPortType=p1  RConnTagsString=__newr0  mask(PV){p2_3q=[100  230], p5q=0.98, p6_7q=[2  -0.5], p8_9q=[1.05  0.95], p10q=1, p11q=on}
      mask prompts: p2_3q "Power and Voltage Ratings [MVA, kV]"; p5q "Voltage Magnitude [p.u.]"; p6_7q "Qmax and Qmin [p.u.  p.u.]"; p8_9q "Vmax and Vmin [p.u.  p.u.]"; p10q "Loss Participation Coefficient"; p11q "Connected"
      mask help:
      | This block defines a static synchronous compensator:
      | P = 0
      | V = Vdes
      mask init:
      | [x,y] = fm_draw('circle');
      | [xc,yc] = fm_draw('C');
      mask CallbackString: |||||fm_block
      mask Display:
      | plot(x,y,[-0.25 -0.25],[-0.25 0.25])
      | color('blue')
      | plot(0.5*xc-0.25,yc)
  Gen115 : fm_lib/Power Flow/PV  Tag=PSATblock  Description=Power Flow  Orientation=down  PhysicalDomain=psatdomain  SubClassName=unknown  LeftPortType=p1  RightPortType=p1  RConnTagsString=__newr0  p2_3q="[100  230]"  p4q=2.15  p5q=1.014  p6_7q="[1.1  -0.5]"  p8_9q="[1.05  0.95]"  p10q=1  p11q=on
  Gen116 : fm_lib/Power Flow/PV  Tag=PSATblock  Description=Power Flow  Orientation=down  PhysicalDomain=psatdomain  SubClassName=unknown  LeftPortType=p1  RightPortType=p1  RConnTagsString=__newr0  p2_3q="[100  230]"  p4q=1.55  p5q=1.017  p6_7q="[0.8  -0.5]"  p8_9q="[1.05  0.95]"  p10q=1  p11q=on
  Gen118 : PMComponent  Tag=PSATblock  Description=Power Flow  Orientation=down  PhysicalDomain=psatdomain  LeftPortType=p1  RightPortType=p1  RConnTagsString=__newr0  mask(PV){p2_3q=[100  230], p4q=4, p5q=1.05, p6_7q=[2  -0.5], p8_9q=[1.05  0.95], p10q=1, p11q=on}
      mask prompts: p2_3q "Power and Voltage Ratings [MVA, kV]"; p4q "Active Power [p.u.]"; p5q "Voltage Magnitude [p.u.]"; p6_7q "Qmax & Qmin [p.u.  p.u.]"; p8_9q "Vmax & Vmin [p.u.  p.u.]"; p10q "Loss Participation Factor"; p11q "Connected"
      mask help:
      | This block defines a PV bus for load flow studies:
      |
      | P = Pcost.
      | V = Vdes.
      mask init:
      | [x,y] = fm_draw('circle');
      | [xp,yp] = fm_draw('P');
      mask CallbackString: ||||||fm_block
      mask Display:
      | plot(x,y)
      | color('blue')
      | plot(0.3*xp-0.35,0.6*yp,[0.1 0.3 0.5],[0.3 -0.3 0.3])
  Gen121 : PMComponent  Tag=PSATblock  Description=Power Flow  Orientation=down  PhysicalDomain=psatdomain  LeftPortType=p1  RightPortType=p1  RConnTagsString=__newr0  mask(PV){p2_3q=[100  230], p4q=4, p5q=1.05, p6_7q=[2  -0.5], p8_9q=[1.05  0.95], p10q=1, p11q=on}
      mask prompts: p2_3q "Power and Voltage Ratings [MVA, kV]"; p4q "Active Power [p.u.]"; p5q "Voltage Magnitude [p.u.]"; p6_7q "Qmax & Qmin [p.u.  p.u.]"; p8_9q "Vmax & Vmin [p.u.  p.u.]"; p10q "Loss Participation Factor"; p11q "Connected"
      mask help:
      | This block defines a PV bus for load flow studies:
      |
      | P = Pcost.
      | V = Vdes.
      mask init:
      | [x,y] = fm_draw('circle');
      | [xp,yp] = fm_draw('P');
      mask CallbackString: ||||||fm_block
      mask Display:
      | plot(x,y)
      | color('blue')
      | plot(0.3*xp-0.35,0.6*yp,[0.1 0.3 0.5],[0.3 -0.3 0.3])
  Gen122 : fm_lib/Power Flow/PV  Tag=PSATblock  Description=Power Flow  Orientation=down  PhysicalDomain=psatdomain  SubClassName=unknown  LeftPortType=p1  RightPortType=p1  RConnTagsString=__newr0  p2_3q="[100  230]"  p4q=3  p5q=1.05  p6_7q="[0.96  -0.6]"  p8_9q="[1.05  0.95]"  p10q=1  p11q=on
  Gen123 : fm_lib/Power Flow/PV  Tag=PSATblock  Description=Power Flow  Orientation=left  PhysicalDomain=psatdomain  SubClassName=unknown  LeftPortType=p1  RightPortType=p1  RConnTagsString=__newr0  p2_3q="[100  230]"  p4q=6.6  p5q=1.05  p6_7q="[3.1  -1.25]"  p8_9q="[1.05  0.95]"  p10q=1  p11q=on
  Load101 : PMComponent  Tag=PSATblock  Description=Power Flow  Orientation=up  PhysicalDomain=psatdomain  LeftPortType=p1  RightPortType=p1  LConnTagsString=__newl0  mask(PQ){p2_3q=[100  138], p4_5q=[1.08  0.22], p6_7q=[1.05  0.95], p8q=on, p9q=on}
      mask prompts: p2_3q "Power and Voltage Ratings [MVA, kV]"; p4_5q "Active and Reactive Powers [p.u.  p.u.]"; p6_7q "Maximum and Minimum Allowable Voltage [p.u.   p.u.]"; p8q "Allow conversion to impendance for min or max voltage"; p9q "Connected"
      mask help:
      | This block defines a constant power load:
      |
      | P = Pcost.
      | Q = Qcost.
      mask CallbackString: |||fm_block|fm_block
      mask Display: plot([1 -0.5 -0.5 1],[0 0.866 -0.866 0])
  Load102 : PMComponent  Tag=PSATblock  Description=Power Flow  Orientation=up  PhysicalDomain=psatdomain  LeftPortType=p1  RightPortType=p1  LConnTagsString=__newl0  mask(PQ){p2_3q=[100  138], p4_5q=[0.97  0.20], p6_7q=[1.05  0.95], p8q=on, p9q=on}
      mask prompts: p2_3q "Power and Voltage Ratings [MVA, kV]"; p4_5q "Active and Reactive Powers [p.u.  p.u.]"; p6_7q "Maximum and Minimum Allowable Voltage [p.u.   p.u.]"; p8q "Allow conversion to impendance for min or max voltage"; p9q "Connected"
      mask help:
      | This block defines a constant power load:
      |
      | P = Pcost.
      | Q = Qcost.
      mask CallbackString: |||fm_block|fm_block
      mask Display: plot([1 -0.5 -0.5 1],[0 0.866 -0.866 0])
  Load103 : PMComponent  Tag=PSATblock  Description=Power Flow  Orientation=left  PhysicalDomain=psatdomain  LeftPortType=p1  RightPortType=p1  LConnTagsString=__newl0  mask(PQ){p2_3q=[100  138], p4_5q=[1.80  0.37], p6_7q=[1.05  0.95], p8q=on, p9q=on}
      mask prompts: p2_3q "Power and Voltage Ratings [MVA, kV]"; p4_5q "Active and Reactive Powers [p.u.  p.u.]"; p6_7q "Maximum and Minimum Allowable Voltage [p.u.   p.u.]"; p8q "Allow conversion to impendance for min or max voltage"; p9q "Connected"
      mask help:
      | This block defines a constant power load:
      |
      | P = Pcost.
      | Q = Qcost.
      mask CallbackString: |||fm_block|fm_block
      mask Display: plot([1 -0.5 -0.5 1],[0 0.866 -0.866 0])
  Load104 : PMComponent  Tag=PSATblock  Description=Power Flow  Orientation=left  PhysicalDomain=psatdomain  LeftPortType=p1  RightPortType=p1  LConnTagsString=__newl0  mask(PQ){p2_3q=[100  138], p4_5q=[0.74  0.15], p6_7q=[1.05  0.95], p8q=on, p9q=on}
      mask prompts: p2_3q "Power and Voltage Ratings [MVA, kV]"; p4_5q "Active and Reactive Powers [p.u.  p.u.]"; p6_7q "Maximum and Minimum Allowable Voltage [p.u.   p.u.]"; p8q "Allow conversion to impendance for min or max voltage"; p9q "Connected"
      mask help:
      | This block defines a constant power load:
      |
      | P = Pcost.
      | Q = Qcost.
      mask CallbackString: |||fm_block|fm_block
      mask Display: plot([1 -0.5 -0.5 1],[0 0.866 -0.866 0])
  Load105 : PMComponent  Tag=PSATblock  Description=Power Flow  Orientation=down  PhysicalDomain=psatdomain  LeftPortType=p1  RightPortType=p1  LConnTagsString=__newl0  mask(PQ){p2_3q=[100  138], p4_5q=[0.71  0.14], p6_7q=[1.05  0.95], p8q=on, p9q=on}
      mask prompts: p2_3q "Power and Voltage Ratings [MVA, kV]"; p4_5q "Active and Reactive Powers [p.u.  p.u.]"; p6_7q "Maximum and Minimum Allowable Voltage [p.u.   p.u.]"; p8q "Allow conversion to impendance for min or max voltage"; p9q "Connected"
      mask help:
      | This block defines a constant power load:
      |
      | P = Pcost.
      | Q = Qcost.
      mask CallbackString: |||fm_block|fm_block
      mask Display: plot([1 -0.5 -0.5 1],[0 0.866 -0.866 0])
  Load106 : PMComponent  Tag=PSATblock  Description=Power Flow  PhysicalDomain=psatdomain  LeftPortType=p1  RightPortType=p1  LConnTagsString=__newl0  mask(PQ){p2_3q=[100  138], p4_5q=[1.36  0.28], p6_7q=[1.05  0.95], p8q=on, p9q=on}
      mask prompts: p2_3q "Power and Voltage Ratings [MVA, kV]"; p4_5q "Active and Reactive Powers [p.u.  p.u.]"; p6_7q "Maximum and Minimum Allowable Voltage [p.u.   p.u.]"; p8q "Allow conversion to impendance for min or max voltage"; p9q "Connected"
      mask help:
      | This block defines a constant power load:
      |
      | P = Pcost.
      | Q = Qcost.
      mask CallbackString: |||fm_block|fm_block
      mask Display: plot([1 -0.5 -0.5 1],[0 0.866 -0.866 0])
  Load107 : PMComponent  Tag=PSATblock  Description=Power Flow  Orientation=up  PhysicalDomain=psatdomain  LeftPortType=p1  RightPortType=p1  LConnTagsString=__newl0  mask(PQ){p2_3q=[100  138], p4_5q=[1.25  0.25], p6_7q=[1.05  0.95], p8q=on, p9q=on}
      mask prompts: p2_3q "Power and Voltage Ratings [MVA, kV]"; p4_5q "Active and Reactive Powers [p.u.  p.u.]"; p6_7q "Maximum and Minimum Allowable Voltage [p.u.   p.u.]"; p8q "Allow conversion to impendance for min or max voltage"; p9q "Connected"
      mask help:
      | This block defines a constant power load:
      |
      | P = Pcost.
      | Q = Qcost.
      mask CallbackString: |||fm_block|fm_block
      mask Display: plot([1 -0.5 -0.5 1],[0 0.866 -0.866 0])
  Load108 : PMComponent  Tag=PSATblock  Description=Power Flow  PhysicalDomain=psatdomain  LeftPortType=p1  RightPortType=p1  LConnTagsString=__newl0  mask(PQ){p2_3q=[100  138], p4_5q=[1.71  0.35], p6_7q=[1.05  0.95], p8q=on, p9q=on}
      mask prompts: p2_3q "Power and Voltage Ratings [MVA, kV]"; p4_5q "Active and Reactive Powers [p.u.  p.u.]"; p6_7q "Maximum and Minimum Allowable Voltage [p.u.   p.u.]"; p8q "Allow conversion to impendance for min or max voltage"; p9q "Connected"
      mask help:
      | This block defines a constant power load:
      |
      | P = Pcost.
      | Q = Qcost.
      mask CallbackString: |||fm_block|fm_block
      mask Display: plot([1 -0.5 -0.5 1],[0 0.866 -0.866 0])
  Load109 : PMComponent  Tag=PSATblock  Description=Power Flow  Orientation=down  PhysicalDomain=psatdomain  LeftPortType=p1  RightPortType=p1  LConnTagsString=__newl0  mask(PQ){p2_3q=[100  138], p4_5q=[1.75  0.36], p6_7q=[1.05  0.95], p8q=on, p9q=on}
      mask prompts: p2_3q "Power and Voltage Ratings [MVA, kV]"; p4_5q "Active and Reactive Powers [p.u.  p.u.]"; p6_7q "Maximum and Minimum Allowable Voltage [p.u.   p.u.]"; p8q "Allow conversion to impendance for min or max voltage"; p9q "Connected"
      mask help:
      | This block defines a constant power load:
      |
      | P = Pcost.
      | Q = Qcost.
      mask CallbackString: |||fm_block|fm_block
      mask Display: plot([1 -0.5 -0.5 1],[0 0.866 -0.866 0])
  Load110 : PMComponent  Tag=PSATblock  Description=Power Flow  Orientation=down  PhysicalDomain=psatdomain  LeftPortType=p1  RightPortType=p1  LConnTagsString=__newl0  mask(PQ){p2_3q=[100  138], p4_5q=[1.95  0.40], p6_7q=[1.05  0.95], p8q=on, p9q=on}
      mask prompts: p2_3q "Power and Voltage Ratings [MVA, kV]"; p4_5q "Active and Reactive Powers [p.u.  p.u.]"; p6_7q "Maximum and Minimum Allowable Voltage [p.u.   p.u.]"; p8q "Allow conversion to impendance for min or max voltage"; p9q "Connected"
      mask help:
      | This block defines a constant power load:
      |
      | P = Pcost.
      | Q = Qcost.
      mask CallbackString: |||fm_block|fm_block
      mask Display: plot([1 -0.5 -0.5 1],[0 0.866 -0.866 0])
  Load113 : PMComponent  Tag=PSATblock  Description=Power Flow  Orientation=left  PhysicalDomain=psatdomain  LeftPortType=p1  RightPortType=p1  LConnTagsString=__newl0  mask(PQ){p2_3q=[100  230], p4_5q=[2.65  0.54], p6_7q=[1.05  0.95], p8q=on, p9q=on}
      mask prompts: p2_3q "Power and Voltage Ratings [MVA, kV]"; p4_5q "Active and Reactive Powers [p.u.  p.u.]"; p6_7q "Maximum and Minimum Allowable Voltage [p.u.   p.u.]"; p8q "Allow conversion to impendance for min or max voltage"; p9q "Connected"
      mask help:
      | This block defines a constant power load:
      |
      | P = Pcost.
      | Q = Qcost.
      mask CallbackString: |||fm_block|fm_block
      mask Display: plot([1 -0.5 -0.5 1],[0 0.866 -0.866 0])
  Load114 : PMComponent  Tag=PSATblock  Description=Power Flow  PhysicalDomain=psatdomain  LeftPortType=p1  RightPortType=p1  LConnTagsString=__newl0  mask(PQ){p2_3q=[100  230], p4_5q=[1.94  0.39], p6_7q=[1.05  0.95], p8q=on, p9q=on}
      mask prompts: p2_3q "Power and Voltage Ratings [MVA, kV]"; p4_5q "Active and Reactive Powers [p.u.  p.u.]"; p6_7q "Maximum and Minimum Allowable Voltage [p.u.   p.u.]"; p8q "Allow conversion to impendance for min or max voltage"; p9q "Connected"
      mask help:
      | This block defines a constant power load:
      |
      | P = Pcost.
      | Q = Qcost.
      mask CallbackString: |||fm_block|fm_block
      mask Display: plot([1 -0.5 -0.5 1],[0 0.866 -0.866 0])
  Load115 : PMComponent  Tag=PSATblock  Description=Power Flow  Orientation=down  PhysicalDomain=psatdomain  LeftPortType=p1  RightPortType=p1  LConnTagsString=__newl0  mask(PQ){p2_3q=[100  230], p4_5q=[3.17  0.64], p6_7q=[1.05  0.95], p8q=on, p9q=on}
      mask prompts: p2_3q "Power and Voltage Ratings [MVA, kV]"; p4_5q "Active and Reactive Powers [p.u.  p.u.]"; p6_7q "Maximum and Minimum Allowable Voltage [p.u.   p.u.]"; p8q "Allow conversion to impendance for min or max voltage"; p9q "Connected"
      mask help:
      | This block defines a constant power load:
      |
      | P = Pcost.
      | Q = Qcost.
      mask CallbackString: |||fm_block|fm_block
      mask Display: plot([1 -0.5 -0.5 1],[0 0.866 -0.866 0])
  Load116 : PMComponent  Tag=PSATblock  Description=Power Flow  Orientation=down  PhysicalDomain=psatdomain  LeftPortType=p1  RightPortType=p1  LConnTagsString=__newl0  mask(PQ){p2_3q=[100  230], p4_5q=[1.0  0.20], p6_7q=[1.05  0.95], p8q=on, p9q=on}
      mask prompts: p2_3q "Power and Voltage Ratings [MVA, kV]"; p4_5q "Active and Reactive Powers [p.u.  p.u.]"; p6_7q "Maximum and Minimum Allowable Voltage [p.u.   p.u.]"; p8q "Allow conversion to impendance for min or max voltage"; p9q "Connected"
      mask help:
      | This block defines a constant power load:
      |
      | P = Pcost.
      | Q = Qcost.
      mask CallbackString: |||fm_block|fm_block
      mask Display: plot([1 -0.5 -0.5 1],[0 0.866 -0.866 0])
  Load118 : PMComponent  Tag=PSATblock  Description=Power Flow  Orientation=down  PhysicalDomain=psatdomain  LeftPortType=p1  RightPortType=p1  LConnTagsString=__newl0  mask(PQ){p2_3q=[100  230], p4_5q=[3.33 0.68], p6_7q=[1.05  0.95], p8q=on, p9q=on}
      mask prompts: p2_3q "Power and Voltage Ratings [MVA, kV]"; p4_5q "Active and Reactive Powers [p.u.  p.u.]"; p6_7q "Maximum and Minimum Allowable Voltage [p.u.   p.u.]"; p8q "Allow conversion to impendance for min or max voltage"; p9q "Connected"
      mask help:
      | This block defines a constant power load:
      |
      | P = Pcost.
      | Q = Qcost.
      mask CallbackString: |||fm_block|fm_block
      mask Display: plot([1 -0.5 -0.5 1],[0 0.866 -0.866 0])
  Load119 : PMComponent  Tag=PSATblock  Description=Power Flow  Orientation=up  PhysicalDomain=psatdomain  LeftPortType=p1  RightPortType=p1  LConnTagsString=__newl0  mask(PQ){p2_3q=[100  230], p4_5q=[1.81  0.37], p6_7q=[1.05  0.95], p8q=on, p9q=on}
      mask prompts: p2_3q "Power and Voltage Ratings [MVA, kV]"; p4_5q "Active and Reactive Powers [p.u.  p.u.]"; p6_7q "Maximum and Minimum Allowable Voltage [p.u.   p.u.]"; p8q "Allow conversion to impendance for min or max voltage"; p9q "Connected"
      mask help:
      | This block defines a constant power load:
      |
      | P = Pcost.
      | Q = Qcost.
      mask CallbackString: |||fm_block|fm_block
      mask Display: plot([1 -0.5 -0.5 1],[0 0.866 -0.866 0])
  Load120 : PMComponent  Tag=PSATblock  Description=Power Flow  Orientation=down  PhysicalDomain=psatdomain  LeftPortType=p1  RightPortType=p1  LConnTagsString=__newl0  mask(PQ){p2_3q=[100  230], p4_5q=[1.28  0.26], p6_7q=[1.05  0.95], p8q=on, p9q=on}
      mask prompts: p2_3q "Power and Voltage Ratings [MVA, kV]"; p4_5q "Active and Reactive Powers [p.u.  p.u.]"; p6_7q "Maximum and Minimum Allowable Voltage [p.u.   p.u.]"; p8q "Allow conversion to impendance for min & max voltage"; p9q "Connected"
      mask help:
      | This block defines a constant power load:
      |
      | P = Pcost.
      | Q = Qcost.
      mask CallbackString: |||fm_block|fm_block
      mask Display: plot([1 -0.5 -0.5 1],[0 0.866 -0.866 0])
  Shunt106 : PMComponent  Tag=PSATblock  Description=Power Flow  Orientation=down  PhysicalDomain=psatdomain  LeftPortType=p1  RightPortType=p1  LConnTagsString=__newl0  mask(Shunt){p2_3_4q=[100  138  60], p6q=-1, p7q=on}
      mask prompts: p2_3_4q "Power, Voltage and Frequency Ratings [MVA, kV, Hz]"; p6q "Susceptance B [p.u.]"; p7q "Connected"
      mask help:
      | This block defines a static condenser:
      |
      | Q = B * V^2
      |
      | (Negative values of B define an inductive load).
      mask init:
      | fm_block
      mask Display: plot(-[0 23 23 24 28 34 40 47 52 55 56 54 51 51 47 46 48 51 57 64 70 75 79 79 77 74 74 70 69 71 75 80 87 93 99 102 103 101 97 97 94 93 94 98 104 110 117 122 125 126 126 150]/150,[0 0 1 11 19 24 25 23 17 8 -2 -12 -18 -18 -9 1 11 19 24 25 23 17 8 -2 -12 -18 -18 -9 1 11 19 24 25 23 17 8 -2 -12 -18 -18 -9 1 11 19 24 25 23 17 8 0 0 0]/45,[0 0],[-0.4 0.4],[0.075 0.075],[-0.25 0.25],[0.15 0.15],[-0.1 0.1],0,-0.5)
  Sup101a : PMComponent  Tag=PSATblock  Description=OPF & CPF  Orientation=up  PhysicalDomain=psatdomain  LeftPortType=p1  RightPortType=p1  RConnTagsString=__newr0  mask(Supply){p2q=100, p3q=0.1, p4_5q=[0.2 0.1], p7_8_9q=[0.0172*100  24.8415  36.505/100], p10_11_12q=[0.00  0.00  0.00], p13q=off, p14q=0, p15q=1, p16_17q=[0.1  0], p18_19q=[0 0], in=0, p20q=on}
      mask prompts: p2q "Power Rating [MVA]"; p3q "Active Power [p.u.]"; p4_5q "Max and Min Power Supply [p.u.  p.u.]"; p7_8_9q "Cost = a + b*P + c*P^2 [$/h, $/MWh, $/(MW)^2 h]"; p10_11_12q "Cost = a + b*Q + c*Q^2 [$/h, $/MVArh, $/(MVAr)^2 h]"; p13q "Allow Unit Commitment"; p14q "Tie Breaking Cost [$/h]"; p15q "Loss participation factor"; p16_17q "Reactive power limits Qmax and Qmin [p.u. p.u.]"; p18_19q "Up and down congestion costs [$/h $/h]"; in "Number of Input Signals"; p20q "Connected"
      mask help: This block defines a PV bus for bifurcation and market studies:
      mask init:
      | fm_inout;
      | [x,y] = fm_draw('circle');
      | [xs,ys] = fm_draw('$');
      mask StyleString: edit,edit,edit,edit,edit,checkbox,edit,edit,edit,edit,popup(0|1|2),checkbox
      mask CallbackString: |||||||||||fm_block
      mask Display:
      | plot(x,y)
      | color('blue')
      | plot(xs,ys)
  Sup101b : PMComponent  Tag=PSATblock  Description=OPF & CPF  Orientation=up  PhysicalDomain=psatdomain  LeftPortType=p1  RightPortType=p1  RConnTagsString=__newr0  mask(Supply){p2q=100, p3q=0.1, p4_5q=[0.2 0.1], p7_8_9q=[0.0172*100  24.8415  36.505/100], p10_11_12q=[0.00  0.00  0.00], p13q=off, p14q=0, p15q=1, p16_17q=[0.1  0], p18_19q=[0 0], in=0, p20q=on}
      mask prompts: p2q "Power Rating [MVA]"; p3q "Active Power [p.u.]"; p4_5q "Max and Min Power Supply [p.u.  p.u.]"; p7_8_9q "Cost = a + b*P + c*P^2 [$/h, $/MWh, $/(MW)^2 h]"; p10_11_12q "Cost = a + b*Q + c*Q^2 [$/h, $/MVArh, $/(MVAr)^2 h]"; p13q "Allow Unit Commitment"; p14q "Tie Breaking Cost [$/h]"; p15q "Loss participation factor"; p16_17q "Reactive power limits Qmax and Qmin [p.u. p.u.]"; p18_19q "Up and down congestion costs [$/h $/h]"; in "Number of Input Signals"; p20q "Connected"
      mask help: This block defines a PV bus for bifurcation and market studies:
      mask init:
      | fm_inout;
      | [x,y] = fm_draw('circle');
      | [xs,ys] = fm_draw('$');
      mask StyleString: edit,edit,edit,edit,edit,checkbox,edit,edit,edit,edit,popup(0|1|2),checkbox
      mask CallbackString: |||||||||||fm_block
      mask Display:
      | plot(x,y)
      | color('blue')
      | plot(xs,ys)
  Sup101c : PMComponent  Tag=PSATblock  Description=OPF & CPF  Orientation=up  PhysicalDomain=psatdomain  LeftPortType=p1  RightPortType=p1  RConnTagsString=__newr0  mask(Supply){p2q=100, p3q=0.76, p4_5q=[0.76 0.152], p7_8_9q=[0.035*100  10.2386  3.8404/100], p10_11_12q=[0.00  0.00  0.00], p13q=off, p14q=0, p15q=1, p16_17q=[0.3  -0.25], p18_19q=[0 0], in=0, p20q=on}
      mask prompts: p2q "Power Rating [MVA]"; p3q "Active Power [p.u.]"; p4_5q "Max and Min Power Supply [p.u.  p.u.]"; p7_8_9q "Cost = a + b*P + c*P^2 [$/h, $/MWh, $/(MW)^2 h]"; p10_11_12q "Cost = a + b*Q + c*Q^2 [$/h, $/MVArh, $/(MVAr)^2 h]"; p13q "Allow Unit Commitment"; p14q "Tie Breaking Cost [$/h]"; p15q "Loss participation factor"; p16_17q "Reactive power limits Qmax and Qmin [p.u. p.u.]"; p18_19q "Up and down congestion costs [$/h $/h]"; in "Number of Input Signals"; p20q "Connected"
      mask help: This block defines a PV bus for bifurcation and market studies:
      mask init:
      | fm_inout;
      | [x,y] = fm_draw('circle');
      | [xs,ys] = fm_draw('$');
      mask StyleString: edit,edit,edit,edit,edit,checkbox,edit,edit,edit,edit,popup(0|1|2),checkbox
      mask CallbackString: |||||||||||fm_block
      mask Display:
      | plot(x,y)
      | color('blue')
      | plot(xs,ys)
  Sup101d : PMComponent  Tag=PSATblock  Description=OPF & CPF  Orientation=up  PhysicalDomain=psatdomain  LeftPortType=p1  RightPortType=p1  RConnTagsString=__newr0  mask(Supply){p2q=100, p3q=0.76, p4_5q=[0.76 0.152], p7_8_9q=[0.035*100  10.2386  3.8404/100], p10_11_12q=[0.00  0.00  0.00], p13q=off, p14q=0, p15q=1, p16_17q=[0.3  -0.25], p18_19q=[0 0], in=0, p20q=on}
      mask prompts: p2q "Power Rating [MVA]"; p3q "Active Power [p.u.]"; p4_5q "Max and Min Power Supply [p.u.  p.u.]"; p7_8_9q "Cost = a + b*P + c*P^2 [$/h, $/MWh, $/(MW)^2 h]"; p10_11_12q "Cost = a + b*Q + c*Q^2 [$/h, $/MVArh, $/(MVAr)^2 h]"; p13q "Allow Unit Commitment"; p14q "Tie Breaking Cost [$/h]"; p15q "Loss participation factor"; p16_17q "Reactive power limits Qmax and Qmin [p.u. p.u.]"; p18_19q "Up and down congestion costs [$/h $/h]"; in "Number of Input Signals"; p20q "Connected"
      mask help: This block defines a PV bus for bifurcation and market studies:
      mask init:
      | fm_inout;
      | [x,y] = fm_draw('circle');
      | [xs,ys] = fm_draw('$');
      mask StyleString: edit,edit,edit,edit,edit,checkbox,edit,edit,edit,edit,popup(0|1|2),checkbox
      mask CallbackString: |||||||||||fm_block
      mask Display:
      | plot(x,y)
      | color('blue')
      | plot(xs,ys)
  Sup102a : PMComponent  Tag=PSATblock  Description=OPF & CPF  Orientation=up  PhysicalDomain=psatdomain  LeftPortType=p1  RightPortType=p1  RConnTagsString=__newr0  mask(Supply){p2q=100, p3q=0.1, p4_5q=[0.2 0.1], p7_8_9q=[0.0172*100  24.8415  36.505/100], p10_11_12q=[0.00  0.00  0.00], p13q=off, p14q=0, p15q=1, p16_17q=[0.1  0], p18_19q=[0 0], in=0, p20q=on}
      mask prompts: p2q "Power Rating [MVA]"; p3q "Active Power [p.u.]"; p4_5q "Max and Min Power Supply [p.u.  p.u.]"; p7_8_9q "Cost = a + b*P + c*P^2 [$/h, $/MWh, $/(MW)^2 h]"; p10_11_12q "Cost = a + b*Q + c*Q^2 [$/h, $/MVArh, $/(MVAr)^2 h]"; p13q "Allow Unit Commitment"; p14q "Tie Breaking Cost [$/h]"; p15q "Loss participation factor"; p16_17q "Reactive power limits Qmax and Qmin [p.u. p.u.]"; p18_19q "Up and down congestion costs [$/h $/h]"; in "Number of Input Signals"; p20q "Connected"
      mask help: This block defines a PV bus for bifurcation and market studies:
      mask init:
      | fm_inout;
      | [x,y] = fm_draw('circle');
      | [xs,ys] = fm_draw('$');
      mask StyleString: edit,edit,edit,edit,edit,checkbox,edit,edit,edit,edit,popup(0|1|2),checkbox
      mask CallbackString: |||||||||||fm_block
      mask Display:
      | plot(x,y)
      | color('blue')
      | plot(xs,ys)
  Sup102b : PMComponent  Tag=PSATblock  Description=OPF & CPF  Orientation=up  PhysicalDomain=psatdomain  LeftPortType=p1  RightPortType=p1  RConnTagsString=__newr0  mask(Supply){p2q=100, p3q=0.1, p4_5q=[0.2 0.1], p7_8_9q=[0.0172*100  24.8415  36.505/100], p10_11_12q=[0.00  0.00  0.00], p13q=off, p14q=0, p15q=1, p16_17q=[0.1  0], p18_19q=[0 0], in=0, p20q=on}
      mask prompts: p2q "Power Rating [MVA]"; p3q "Active Power [p.u.]"; p4_5q "Max and Min Power Supply [p.u.  p.u.]"; p7_8_9q "Cost = a + b*P + c*P^2 [$/h, $/MWh, $/(MW)^2 h]"; p10_11_12q "Cost = a + b*Q + c*Q^2 [$/h, $/MVArh, $/(MVAr)^2 h]"; p13q "Allow Unit Commitment"; p14q "Tie Breaking Cost [$/h]"; p15q "Loss participation factor"; p16_17q "Reactive power limits Qmax and Qmin [p.u. p.u.]"; p18_19q "Up and down congestion costs [$/h $/h]"; in "Number of Input Signals"; p20q "Connected"
      mask help: This block defines a PV bus for bifurcation and market studies:
      mask init:
      | fm_inout;
      | [x,y] = fm_draw('circle');
      | [xs,ys] = fm_draw('$');
      mask StyleString: edit,edit,edit,edit,edit,checkbox,edit,edit,edit,edit,popup(0|1|2),checkbox
      mask CallbackString: |||||||||||fm_block
      mask Display:
      | plot(x,y)
      | color('blue')
      | plot(xs,ys)
  Sup102c : PMComponent  Tag=PSATblock  Description=OPF & CPF  Orientation=up  PhysicalDomain=psatdomain  LeftPortType=p1  RightPortType=p1  RConnTagsString=__newr0  mask(Supply){p2q=100, p3q=0.76, p4_5q=[0.76 0.152], p7_8_9q=[0.035*100  10.2386  3.8404/100], p10_11_12q=[0.00  0.00  0.00], p13q=off, p14q=0, p15q=1, p16_17q=[0.3  -0.25], p18_19q=[0 0], in=0, p20q=on}
      mask prompts: p2q "Power Rating [MVA]"; p3q "Active Power [p.u.]"; p4_5q "Max and Min Power Supply [p.u.  p.u.]"; p7_8_9q "Cost = a + b*P + c*P^2 [$/h, $/MWh, $/(MW)^2 h]"; p10_11_12q "Cost = a + b*Q + c*Q^2 [$/h, $/MVArh, $/(MVAr)^2 h]"; p13q "Allow Unit Commitment"; p14q "Tie Breaking Cost [$/h]"; p15q "Loss participation factor"; p16_17q "Reactive power limits Qmax and Qmin [p.u. p.u.]"; p18_19q "Up and down congestion costs [$/h $/h]"; in "Number of Input Signals"; p20q "Connected"
      mask help: This block defines a PV bus for bifurcation and market studies:
      mask init:
      | fm_inout;
      | [x,y] = fm_draw('circle');
      | [xs,ys] = fm_draw('$');
      mask StyleString: edit,edit,edit,edit,edit,checkbox,edit,edit,edit,edit,popup(0|1|2),checkbox
      mask CallbackString: |||||||||||fm_block
      mask Display:
      | plot(x,y)
      | color('blue')
      | plot(xs,ys)
  Sup102d : PMComponent  Tag=PSATblock  Description=OPF & CPF  Orientation=up  PhysicalDomain=psatdomain  LeftPortType=p1  RightPortType=p1  RConnTagsString=__newr0  mask(Supply){p2q=100, p3q=0.76, p4_5q=[0.76 0.152], p7_8_9q=[0.035*100  10.2386  3.8404/100], p10_11_12q=[0.00  0.00  0.00], p13q=off, p14q=0, p15q=1, p16_17q=[0.3  -0.25], p18_19q=[0 0], in=0, p20q=on}
      mask prompts: p2q "Power Rating [MVA]"; p3q "Active Power [p.u.]"; p4_5q "Max and Min Power Supply [p.u.  p.u.]"; p7_8_9q "Cost = a + b*P + c*P^2 [$/h, $/MWh, $/(MW)^2 h]"; p10_11_12q "Cost = a + b*Q + c*Q^2 [$/h, $/MVArh, $/(MVAr)^2 h]"; p13q "Allow Unit Commitment"; p14q "Tie Breaking Cost [$/h]"; p15q "Loss participation factor"; p16_17q "Reactive power limits Qmax and Qmin [p.u. p.u.]"; p18_19q "Up and down congestion costs [$/h $/h]"; in "Number of Input Signals"; p20q "Connected"
      mask help: This block defines a PV bus for bifurcation and market studies:
      mask init:
      | fm_inout;
      | [x,y] = fm_draw('circle');
      | [xs,ys] = fm_draw('$');
      mask StyleString: edit,edit,edit,edit,edit,checkbox,edit,edit,edit,edit,popup(0|1|2),checkbox
      mask CallbackString: |||||||||||fm_block
      mask Display:
      | plot(x,y)
      | color('blue')
      | plot(xs,ys)
  Sup107a : PMComponent  Tag=PSATblock  Description=OPF & CPF  Orientation=up  PhysicalDomain=psatdomain  LeftPortType=p1  RightPortType=p1  RConnTagsString=__newr0  mask(Supply){p2q=100, p3q=0.8, p4_5q=[1.00  0.25], p7_8_9q=[-0.0065*100  17.9744  2.7484/100], p10_11_12q=[0.00  0.00  0.00], p13q=off, p14q=0, p15q=1, p16_17q=[0.6  0], p18_19q=[0 0], in=0, p20q=on}
      mask prompts: p2q "Power Rating [MVA]"; p3q "Active Power [p.u.]"; p4_5q "Max and Min Power Supply [p.u.  p.u.]"; p7_8_9q "Cost = a + b*P + c*P^2 [$/h, $/MWh, $/(MW)^2 h]"; p10_11_12q "Cost = a + b*Q + c*Q^2 [$/h, $/MVArh, $/(MVAr)^2 h]"; p13q "Allow Unit Commitment"; p14q "Tie Breaking Cost [$/h]"; p15q "Loss participation factor"; p16_17q "Reactive power limits Qmax and Qmin [p.u. p.u.]"; p18_19q "Up and down congestion costs [$/h $/h]"; in "Number of Input Signals"; p20q "Connected"
      mask help: This block defines a PV bus for bifurcation and market studies:
      mask init:
      | fm_inout;
      | [x,y] = fm_draw('circle');
      | [xs,ys] = fm_draw('$');
      mask StyleString: edit,edit,edit,edit,edit,checkbox,edit,edit,edit,edit,popup(0|1|2),checkbox
      mask CallbackString: |||||||||||fm_block
      mask Display:
      | plot(x,y)
      | color('blue')
      | plot(xs,ys)
  Sup107b : PMComponent  Tag=PSATblock  Description=OPF & CPF  Orientation=up  PhysicalDomain=psatdomain  LeftPortType=p1  RightPortType=p1  RConnTagsString=__newr0  mask(Supply){p2q=100, p3q=0.8, p4_5q=[1.00  0.25], p7_8_9q=[-0.0065*100  17.9744  2.7484/100], p10_11_12q=[0.00  0.00  0.00], p13q=off, p14q=0, p15q=1, p16_17q=[0.6   0], p18_19q=[0 0], in=0, p20q=on}
      mask prompts: p2q "Power Rating [MVA]"; p3q "Active Power [p.u.]"; p4_5q "Max and Min Power Supply [p.u.  p.u.]"; p7_8_9q "Cost = a + b*P + c*P^2 [$/h, $/MWh, $/(MW)^2 h]"; p10_11_12q "Cost = a + b*Q + c*Q^2 [$/h, $/MVArh, $/(MVAr)^2 h]"; p13q "Allow Unit Commitment"; p14q "Tie Breaking Cost [$/h]"; p15q "Loss participation factor"; p16_17q "Reactive power limits Qmax and Qmin [p.u. p.u.]"; p18_19q "Up and down congestion costs [$/h $/h]"; in "Number of Input Signals"; p20q "Connected"
      mask help: This block defines a PV bus for bifurcation and market studies:
      mask init:
      | fm_inout;
      | [x,y] = fm_draw('circle');
      | [xs,ys] = fm_draw('$');
      mask StyleString: edit,edit,edit,edit,edit,checkbox,edit,edit,edit,edit,popup(0|1|2),checkbox
      mask CallbackString: |||||||||||fm_block
      mask Display:
      | plot(x,y)
      | color('blue')
      | plot(xs,ys)
  Sup107c : PMComponent  Tag=PSATblock  Description=OPF & CPF  Orientation=up  PhysicalDomain=psatdomain  LeftPortType=p1  RightPortType=p1  RConnTagsString=__newr0  mask(Supply){p2q=100, p3q=0.8, p4_5q=[1.00  0.25], p7_8_9q=[-0.0065*100  17.9744  2.7484/100], p10_11_12q=[0.00  0.00  0.00], p13q=off, p14q=0, p15q=1, p16_17q=[0.6  0], p18_19q=[0 0], in=0, p20q=on}
      mask prompts: p2q "Power Rating [MVA]"; p3q "Active Power [p.u.]"; p4_5q "Max and Min Power Supply [p.u.  p.u.]"; p7_8_9q "Cost = a + b*P + c*P^2 [$/h, $/MWh, $/(MW)^2 h]"; p10_11_12q "Cost = a + b*Q + c*Q^2 [$/h, $/MVArh, $/(MVAr)^2 h]"; p13q "Allow Unit Commitment"; p14q "Tie Breaking Cost [$/h]"; p15q "Loss participation factor"; p16_17q "Reactive power limits Qmax and Qmin [p.u. p.u.]"; p18_19q "Up and down congestion costs [$/h $/h]"; in "Number of Input Signals"; p20q "Connected"
      mask help: This block defines a PV bus for bifurcation and market studies:
      mask init:
      | fm_inout;
      | [x,y] = fm_draw('circle');
      | [xs,ys] = fm_draw('$');
      mask StyleString: edit,edit,edit,edit,edit,checkbox,edit,edit,edit,edit,popup(0|1|2),checkbox
      mask CallbackString: |||||||||||fm_block
      mask Display:
      | plot(x,y)
      | color('blue')
      | plot(xs,ys)
  Sup113a : PMComponent  Tag=PSATblock  Description=OPF & CPF  Orientation=left  PhysicalDomain=psatdomain  LeftPortType=p1  RightPortType=p1  RConnTagsString=__newr0  mask(Supply){p2q=100, p3q=1.5774, p4_5q=[1.97  0.6895], p7_8_9q=[0.0058*100  18.47  1.0109/100], p10_11_12q=[0.00  0.00  0.00], p13q=off, p14q=0, p15q=1, p16_17q=[0.8 0], p18_19q=[0 0], in=0, p20q=on}
      mask prompts: p2q "Power Rating [MVA]"; p3q "Active Power [p.u.]"; p4_5q "Max and Min Power Supply [p.u.  p.u.]"; p7_8_9q "Cost = a + b*P + c*P^2 [$/h, $/MWh, $/(MW)^2 h]"; p10_11_12q "Cost = a + b*Q + c*Q^2 [$/h, $/MVArh, $/(MVAr)^2 h]"; p13q "Allow Unit Commitment"; p14q "Tie Breaking Cost [$/h]"; p15q "Loss participation factor"; p16_17q "Reactive power limits Qmax and Qmin [p.u. p.u.]"; p18_19q "Up and down congestion costs [$/h $/h]"; in "Number of Input Signals"; p20q "Connected"
      mask help: This block defines a PV bus for bifurcation and market studies:
      mask init:
      | fm_inout;
      | [x,y] = fm_draw('circle');
      | [xs,ys] = fm_draw('$');
      mask StyleString: edit,edit,edit,edit,edit,checkbox,edit,edit,edit,edit,popup(0|1|2),checkbox
      mask CallbackString: |||||||||||fm_block
      mask Display:
      | plot(x,y)
      | color('blue')
      | plot(xs,ys)
  Sup113b : PMComponent  Tag=PSATblock  Description=OPF & CPF  Orientation=left  PhysicalDomain=psatdomain  LeftPortType=p1  RightPortType=p1  RConnTagsString=__newr0  mask(Supply){p2q=100, p3q=1.5774, p4_5q=[1.97  0.6895], p7_8_9q=[0.0058*100  18.47  1.0109/100], p10_11_12q=[0.00  0.00  0.00], p13q=off, p14q=0, p15q=1, p16_17q=[0.8 0], p18_19q=[0 0], in=0, p20q=on}
      mask prompts: p2q "Power Rating [MVA]"; p3q "Active Power [p.u.]"; p4_5q "Max and Min Power Supply [p.u.  p.u.]"; p7_8_9q "Cost = a + b*P + c*P^2 [$/h, $/MWh, $/(MW)^2 h]"; p10_11_12q "Cost = a + b*Q + c*Q^2 [$/h, $/MVArh, $/(MVAr)^2 h]"; p13q "Allow Unit Commitment"; p14q "Tie Breaking Cost [$/h]"; p15q "Loss participation factor"; p16_17q "Reactive power limits Qmax and Qmin [p.u. p.u.]"; p18_19q "Up and down congestion costs [$/h $/h]"; in "Number of Input Signals"; p20q "Connected"
      mask help: This block defines a PV bus for bifurcation and market studies:
      mask init:
      | fm_inout;
      | [x,y] = fm_draw('circle');
      | [xs,ys] = fm_draw('$');
      mask StyleString: edit,edit,edit,edit,edit,checkbox,edit,edit,edit,edit,popup(0|1|2),checkbox
      mask CallbackString: |||||||||||fm_block
      mask Display:
      | plot(x,y)
      | color('blue')
      | plot(xs,ys)
  Sup113c : PMComponent  Tag=PSATblock  Description=OPF & CPF  Orientation=left  PhysicalDomain=psatdomain  LeftPortType=p1  RightPortType=p1  RConnTagsString=__newr0  mask(Supply){p2q=100, p3q=1.5774, p4_5q=[1.97  0.6895], p7_8_9q=[0.0058*100  18.47  1.0109/100], p10_11_12q=[0.00  0.00  0.00], p13q=off, p14q=0, p15q=1, p16_17q=[0.8 0], p18_19q=[0 0], in=0, p20q=on}
      mask prompts: p2q "Power Rating [MVA]"; p3q "Active Power [p.u.]"; p4_5q "Max and Min Power Supply [p.u.  p.u.]"; p7_8_9q "Cost = a + b*P + c*P^2 [$/h, $/MWh, $/(MW)^2 h]"; p10_11_12q "Cost = a + b*Q + c*Q^2 [$/h, $/MVArh, $/(MVAr)^2 h]"; p13q "Allow Unit Commitment"; p14q "Tie Breaking Cost [$/h]"; p15q "Loss participation factor"; p16_17q "Reactive power limits Qmax and Qmin [p.u. p.u.]"; p18_19q "Up and down congestion costs [$/h $/h]"; in "Number of Input Signals"; p20q "Connected"
      mask help: This block defines a PV bus for bifurcation and market studies:
      mask init:
      | fm_inout;
      | [x,y] = fm_draw('circle');
      | [xs,ys] = fm_draw('$');
      mask StyleString: edit,edit,edit,edit,edit,checkbox,edit,edit,edit,edit,popup(0|1|2),checkbox
      mask CallbackString: |||||||||||fm_block
      mask Display:
      | plot(x,y)
      | color('blue')
      | plot(xs,ys)
  Sup115a : PMComponent  Tag=PSATblock  Description=OPF & CPF  Orientation=down  PhysicalDomain=psatdomain  LeftPortType=p1  RightPortType=p1  RConnTagsString=__newr0  mask(Supply){p2q=100, p3q=1.55, p4_5q=[1.55  0.5425], p7_8_9q=[0.0109*100  9.5369  0.5586/100], p10_11_12q=[0.00  0.00  0.00], p13q=off, p14q=0, p15q=1, p16_17q=[0.8  -0.5], p18_19q=[0 0], in=0, p20q=on}
      mask prompts: p2q "Power Rating [MVA]"; p3q "Active Power [p.u.]"; p4_5q "Max and Min Power Supply [p.u.  p.u.]"; p7_8_9q "Cost = a + b*P + c*P^2 [$/h, $/MWh, $/(MW)^2 h]"; p10_11_12q "Cost = a + b*Q + c*Q^2 [$/h, $/MVArh, $/(MVAr)^2 h]"; p13q "Allow Unit Commitment"; p14q "Tie Breaking Cost [$/h]"; p15q "Loss participation factor"; p16_17q "Reactive power limits Qmax and Qmin [p.u. p.u.]"; p18_19q "Up and down congestion costs [$/h $/h]"; in "Number of Input Signals"; p20q "Connected"
      mask help: This block defines a PV bus for bifurcation and market studies:
      mask init:
      | fm_inout;
      | [x,y] = fm_draw('circle');
      | [xs,ys] = fm_draw('$');
      mask StyleString: edit,edit,edit,edit,edit,checkbox,edit,edit,edit,edit,popup(0|1|2),checkbox
      mask CallbackString: |||||||||||fm_block
      mask Display:
      | plot(x,y)
      | color('blue')
      | plot(xs,ys)
  Sup115b : PMComponent  Tag=PSATblock  Description=OPF & CPF  Orientation=down  PhysicalDomain=psatdomain  LeftPortType=p1  RightPortType=p1  RConnTagsString=__newr0  mask(Supply){p2q=100, p3q=0.12, p4_5q=[0.12  0.024], p7_8_9q=[0.0111*100  21.2267  37.9372/100], p10_11_12q=[0.00  0.00  0.00], p13q=off, p14q=0, p15q=1, p16_17q=[0.06 0], p18_19q=[0 0], in=0, p20q=on}
      mask prompts: p2q "Power Rating [MVA]"; p3q "Active Power [p.u.]"; p4_5q "Max and Min Power Supply [p.u.  p.u.]"; p7_8_9q "Cost = a + b*P + c*P^2 [$/h, $/MWh, $/(MW)^2 h]"; p10_11_12q "Cost = a + b*Q + c*Q^2 [$/h, $/MVArh, $/(MVAr)^2 h]"; p13q "Allow Unit Commitment"; p14q "Tie Breaking Cost [$/h]"; p15q "Loss participation factor"; p16_17q "Reactive power limits Qmax and Qmin [p.u. p.u.]"; p18_19q "Up and down congestion costs [$/h $/h]"; in "Number of Input Signals"; p20q "Connected"
      mask help: This block defines a PV bus for bifurcation and market studies:
      mask init:
      | fm_inout;
      | [x,y] = fm_draw('circle');
      | [xs,ys] = fm_draw('$');
      mask StyleString: edit,edit,edit,edit,edit,checkbox,edit,edit,edit,edit,popup(0|1|2),checkbox
      mask CallbackString: |||||||||||fm_block
      mask Display:
      | plot(x,y)
      | color('blue')
      | plot(xs,ys)
  Sup115c : PMComponent  Tag=PSATblock  Description=OPF & CPF  Orientation=down  PhysicalDomain=psatdomain  LeftPortType=p1  RightPortType=p1  RConnTagsString=__newr0  mask(Supply){p2q=100, p3q=0.12, p4_5q=[0.12  0.024], p7_8_9q=[0.0111*100  21.2267  37.9372/100], p10_11_12q=[0.00  0.00  0.00], p13q=off, p14q=0, p15q=1, p16_17q=[0.06 0], p18_19q=[0 0], in=0, p20q=on}
      mask prompts: p2q "Power Rating [MVA]"; p3q "Active Power [p.u.]"; p4_5q "Max and Min Power Supply [p.u.  p.u.]"; p7_8_9q "Cost = a + b*P + c*P^2 [$/h, $/MWh, $/(MW)^2 h]"; p10_11_12q "Cost = a + b*Q + c*Q^2 [$/h, $/MVArh, $/(MVAr)^2 h]"; p13q "Allow Unit Commitment"; p14q "Tie Breaking Cost [$/h]"; p15q "Loss participation factor"; p16_17q "Reactive power limits Qmax and Qmin [p.u. p.u.]"; p18_19q "Up and down congestion costs [$/h $/h]"; in "Number of Input Signals"; p20q "Connected"
      mask help: This block defines a PV bus for bifurcation and market studies:
      mask init:
      | fm_inout;
      | [x,y] = fm_draw('circle');
      | [xs,ys] = fm_draw('$');
      mask StyleString: edit,edit,edit,edit,edit,checkbox,edit,edit,edit,edit,popup(0|1|2),checkbox
      mask CallbackString: |||||||||||fm_block
      mask Display:
      | plot(x,y)
      | color('blue')
      | plot(xs,ys)
  Sup115d : PMComponent  Tag=PSATblock  Description=OPF & CPF  Orientation=down  PhysicalDomain=psatdomain  LeftPortType=p1  RightPortType=p1  RConnTagsString=__newr0  mask(Supply){p2q=100, p3q=0.12, p4_5q=[0.12  0.024], p7_8_9q=[0.0111*100  21.2267  37.9372/100], p10_11_12q=[0.00  0.00  0.00], p13q=off, p14q=0, p15q=1, p16_17q=[0.06 0], p18_19q=[0 0], in=0, p20q=on}
      mask prompts: p2q "Power Rating [MVA]"; p3q "Active Power [p.u.]"; p4_5q "Max and Min Power Supply [p.u.  p.u.]"; p7_8_9q "Cost = a + b*P + c*P^2 [$/h, $/MWh, $/(MW)^2 h]"; p10_11_12q "Cost = a + b*Q + c*Q^2 [$/h, $/MVArh, $/(MVAr)^2 h]"; p13q "Allow Unit Commitment"; p14q "Tie Breaking Cost [$/h]"; p15q "Loss participation factor"; p16_17q "Reactive power limits Qmax and Qmin [p.u. p.u.]"; p18_19q "Up and down congestion costs [$/h $/h]"; in "Number of Input Signals"; p20q "Connected"
      mask help: This block defines a PV bus for bifurcation and market studies:
      mask init:
      | fm_inout;
      | [x,y] = fm_draw('circle');
      | [xs,ys] = fm_draw('$');
      mask StyleString: edit,edit,edit,edit,edit,checkbox,edit,edit,edit,edit,popup(0|1|2),checkbox
      mask CallbackString: |||||||||||fm_block
      mask Display:
      | plot(x,y)
      | color('blue')
      | plot(xs,ys)
  Sup115e : PMComponent  Tag=PSATblock  Description=OPF & CPF  Orientation=down  PhysicalDomain=psatdomain  LeftPortType=p1  RightPortType=p1  RConnTagsString=__newr0  mask(Supply){p2q=100, p3q=0.12, p4_5q=[0.12  0.024], p7_8_9q=[0.0111*100  21.2267  37.9372/100], p10_11_12q=[0.00  0.00  0.00], p13q=off, p14q=0, p15q=1, p16_17q=[0.06 0], p18_19q=[0 0], in=0, p20q=on}
      mask prompts: p2q "Power Rating [MVA]"; p3q "Active Power [p.u.]"; p4_5q "Max and Min Power Supply [p.u.  p.u.]"; p7_8_9q "Cost = a + b*P + c*P^2 [$/h, $/MWh, $/(MW)^2 h]"; p10_11_12q "Cost = a + b*Q + c*Q^2 [$/h, $/MVArh, $/(MVAr)^2 h]"; p13q "Allow Unit Commitment"; p14q "Tie Breaking Cost [$/h]"; p15q "Loss participation factor"; p16_17q "Reactive power limits Qmax and Qmin [p.u. p.u.]"; p18_19q "Up and down congestion costs [$/h $/h]"; in "Number of Input Signals"; p20q "Connected"
      mask help: This block defines a PV bus for bifurcation and market studies:
      mask init:
      | fm_inout;
      | [x,y] = fm_draw('circle');
      | [xs,ys] = fm_draw('$');
      mask StyleString: edit,edit,edit,edit,edit,checkbox,edit,edit,edit,edit,popup(0|1|2),checkbox
      mask CallbackString: |||||||||||fm_block
      mask Display:
      | plot(x,y)
      | color('blue')
      | plot(xs,ys)
  Sup115f : PMComponent  Tag=PSATblock  Description=OPF & CPF  Orientation=down  PhysicalDomain=psatdomain  LeftPortType=p1  RightPortType=p1  RConnTagsString=__newr0  mask(Supply){p2q=100, p3q=0.12, p4_5q=[0.12  0.024], p7_8_9q=[0.0111*100  21.2267  37.9372/100], p10_11_12q=[0.00  0.00  0.00], p13q=off, p14q=0, p15q=1, p16_17q=[0.06 0], p18_19q=[0 0], in=0, p20q=on}
      mask prompts: p2q "Power Rating [MVA]"; p3q "Active Power [p.u.]"; p4_5q "Max and Min Power Supply [p.u.  p.u.]"; p7_8_9q "Cost = a + b*P + c*P^2 [$/h, $/MWh, $/(MW)^2 h]"; p10_11_12q "Cost = a + b*Q + c*Q^2 [$/h, $/MVArh, $/(MVAr)^2 h]"; p13q "Allow Unit Commitment"; p14q "Tie Breaking Cost [$/h]"; p15q "Loss participation factor"; p16_17q "Reactive power limits Qmax and Qmin [p.u. p.u.]"; p18_19q "Up and down congestion costs [$/h $/h]"; in "Number of Input Signals"; p20q "Connected"
      mask help: This block defines a PV bus for bifurcation and market studies:
      mask init:
      | fm_inout;
      | [x,y] = fm_draw('circle');
      | [xs,ys] = fm_draw('$');
      mask StyleString: edit,edit,edit,edit,edit,checkbox,edit,edit,edit,edit,popup(0|1|2),checkbox
      mask CallbackString: |||||||||||fm_block
      mask Display:
      | plot(x,y)
      | color('blue')
      | plot(xs,ys)
  Sup116 : PMComponent  Tag=PSATblock  Description=OPF & CPF  Orientation=down  PhysicalDomain=psatdomain  LeftPortType=p1  RightPortType=p1  RConnTagsString=__newr0  mask(Supply){p2q=100, p3q=1.55, p4_5q=[1.55  0.5425], p7_8_9q=[0.0109*100  9.5369  0.5586/100], p10_11_12q=[0.00  0.00  0.00], p13q=off, p14q=0, p15q=1, p16_17q=[0.8   -0.5], p18_19q=[0 0], in=0, p20q=on}
      mask prompts: p2q "Power Rating [MVA]"; p3q "Active Power [p.u.]"; p4_5q "Max and Min Power Supply [p.u.  p.u.]"; p7_8_9q "Cost = a + b*P + c*P^2 [$/h, $/MWh, $/(MW)^2 h]"; p10_11_12q "Cost = a + b*Q + c*Q^2 [$/h, $/MVArh, $/(MVAr)^2 h]"; p13q "Allow Unit Commitment"; p14q "Tie Breaking Cost [$/h]"; p15q "Loss participation factor"; p16_17q "Reactive power limits Qmax and Qmin [p.u. p.u.]"; p18_19q "Up and down congestion costs [$/h $/h]"; in "Number of Input Signals"; p20q "Connected"
      mask help: This block defines a PV bus for bifurcation and market studies:
      mask init:
      | fm_inout;
      | [x,y] = fm_draw('circle');
      | [xs,ys] = fm_draw('$');
      mask StyleString: edit,edit,edit,edit,edit,checkbox,edit,edit,edit,edit,popup(0|1|2),checkbox
      mask CallbackString: |||||||||||fm_block
      mask Display:
      | plot(x,y)
      | color('blue')
      | plot(xs,ys)
  Sup118 : PMComponent  Tag=PSATblock  Description=OPF & CPF  Orientation=down  PhysicalDomain=psatdomain  LeftPortType=p1  RightPortType=p1  RConnTagsString=__newr0  mask(Supply){p2q=100, p3q=4, p4_5q=[4.00 1.00], p7_8_9q=[0.0576*100  5.2301  0.0067/100], p10_11_12q=[0.00  0.00  0.00], p13q=off, p14q=0, p15q=1, p16_17q=[2  -0.5], p18_19q=[0 0], in=0, p20q=on}
      mask prompts: p2q "Power Rating [MVA]"; p3q "Active Power [p.u.]"; p4_5q "Max and Min Power Supply [p.u.  p.u.]"; p7_8_9q "Cost = a + b*P + c*P^2 [$/h, $/MWh, $/(MW)^2 h]"; p10_11_12q "Cost = a + b*Q + c*Q^2 [$/h, $/MVArh, $/(MVAr)^2 h]"; p13q "Allow Unit Commitment"; p14q "Tie Breaking Cost [$/h]"; p15q "Loss participation factor"; p16_17q "Reactive power limits Qmax and Qmin [p.u. p.u.]"; p18_19q "Up and down congestion costs [$/h $/h]"; in "Number of Input Signals"; p20q "Connected"
      mask help: This block defines a PV bus for bifurcation and market studies:
      mask init:
      | fm_inout;
      | [x,y] = fm_draw('circle');
      | [xs,ys] = fm_draw('$');
      mask StyleString: edit,edit,edit,edit,edit,checkbox,edit,edit,edit,edit,popup(0|1|2),checkbox
      mask CallbackString: |||||||||||fm_block
      mask Display:
      | plot(x,y)
      | color('blue')
      | plot(xs,ys)
  Sup121 : PMComponent  Tag=PSATblock  Description=OPF & CPF  Orientation=left  PhysicalDomain=psatdomain  LeftPortType=p1  RightPortType=p1  RConnTagsString=__newr0  mask(Supply){p2q=100, p3q=4, p4_5q=[4.00 1.00], p7_8_9q=[0.0576*100  5.2301  0.0067/100], p10_11_12q=[0.00  0.00  0.00], p13q=off, p14q=0, p15q=1, p16_17q=[2.0   -0.5], p18_19q=[0 0], in=0, p20q=on}
      mask prompts: p2q "Power Rating [MVA]"; p3q "Active Power [p.u.]"; p4_5q "Max and Min Power Supply [p.u.  p.u.]"; p7_8_9q "Cost = a + b*P + c*P^2 [$/h, $/MWh, $/(MW)^2 h]"; p10_11_12q "Cost = a + b*Q + c*Q^2 [$/h, $/MVArh, $/(MVAr)^2 h]"; p13q "Allow Unit Commitment"; p14q "Tie Breaking Cost [$/h]"; p15q "Loss participation factor"; p16_17q "Reactive power limits Qmax and Qmin [p.u. p.u.]"; p18_19q "Up and down congestion costs [$/h $/h]"; in "Number of Input Signals"; p20q "Connected"
      mask help: This block defines a PV bus for bifurcation and market studies:
      mask init:
      | fm_inout;
      | [x,y] = fm_draw('circle');
      | [xs,ys] = fm_draw('$');
      mask StyleString: edit,edit,edit,edit,edit,checkbox,edit,edit,edit,edit,popup(0|1|2),checkbox
      mask CallbackString: |||||||||||fm_block
      mask Display:
      | plot(x,y)
      | color('blue')
      | plot(xs,ys)
  Sup122a : PMComponent  Tag=PSATblock  Description=OPF & CPF  Orientation=down  PhysicalDomain=psatdomain  LeftPortType=p1  RightPortType=p1  RConnTagsString=__newr0  mask(Supply){p2q=100, p3q=0.5, p4_5q=[0.5  0], p7_8_9q=[0.00  1  0.00], p10_11_12q=[0.00  0.00  0.00], p13q=off, p14q=0, p15q=1, p16_17q=[0.16  -0.1], p18_19q=[0 0], in=0, p20q=on}
      mask prompts: p2q "Power Rating [MVA]"; p3q "Active Power [p.u.]"; p4_5q "Max and Min Power Supply [p.u.  p.u.]"; p7_8_9q "Cost = a + b*P + c*P^2 [$/h, $/MWh, $/(MW)^2 h]"; p10_11_12q "Cost = a + b*Q + c*Q^2 [$/h, $/MVArh, $/(MVAr)^2 h]"; p13q "Allow Unit Commitment"; p14q "Tie Breaking Cost [$/h]"; p15q "Loss participation factor"; p16_17q "Reactive power limits Qmax and Qmin [p.u. p.u.]"; p18_19q "Up and down congestion costs [$/h $/h]"; in "Number of Input Signals"; p20q "Connected"
      mask help: This block defines a PV bus for bifurcation and market studies:
      mask init:
      | fm_inout;
      | [x,y] = fm_draw('circle');
      | [xs,ys] = fm_draw('$');
      mask StyleString: edit,edit,edit,edit,edit,checkbox,edit,edit,edit,edit,popup(0|1|2),checkbox
      mask CallbackString: |||||||||||fm_block
      mask Display:
      | plot(x,y)
      | color('blue')
      | plot(xs,ys)
  Sup122b : PMComponent  Tag=PSATblock  Description=OPF & CPF  Orientation=down  PhysicalDomain=psatdomain  LeftPortType=p1  RightPortType=p1  RConnTagsString=__newr0  mask(Supply){p2q=100, p3q=0.5, p4_5q=[0.5  0], p7_8_9q=[0.00  1  0.00], p10_11_12q=[0.00  0.00  0.00], p13q=off, p14q=0, p15q=1, p16_17q=[0.16  -0.1], p18_19q=[0 0], in=0, p20q=on}
      mask prompts: p2q "Power Rating [MVA]"; p3q "Active Power [p.u.]"; p4_5q "Max and Min Power Supply [p.u.  p.u.]"; p7_8_9q "Cost = a + b*P + c*P^2 [$/h, $/MWh, $/(MW)^2 h]"; p10_11_12q "Cost = a + b*Q + c*Q^2 [$/h, $/MVArh, $/(MVAr)^2 h]"; p13q "Allow Unit Commitment"; p14q "Tie Breaking Cost [$/h]"; p15q "Loss participation factor"; p16_17q "Reactive power limits Qmax and Qmin [p.u. p.u.]"; p18_19q "Up and down congestion costs [$/h $/h]"; in "Number of Input Signals"; p20q "Connected"
      mask help: This block defines a PV bus for bifurcation and market studies:
      mask init:
      | fm_inout;
      | [x,y] = fm_draw('circle');
      | [xs,ys] = fm_draw('$');
      mask StyleString: edit,edit,edit,edit,edit,checkbox,edit,edit,edit,edit,popup(0|1|2),checkbox
      mask CallbackString: |||||||||||fm_block
      mask Display:
      | plot(x,y)
      | color('blue')
      | plot(xs,ys)
  Sup122c : PMComponent  Tag=PSATblock  Description=OPF & CPF  Orientation=down  PhysicalDomain=psatdomain  LeftPortType=p1  RightPortType=p1  RConnTagsString=__newr0  mask(Supply){p2q=100, p3q=0.5, p4_5q=[0.5  0], p7_8_9q=[0.00  1  0.00], p10_11_12q=[0.00  0.00  0.00], p13q=off, p14q=0, p15q=1, p16_17q=[0.16  -0.1], p18_19q=[0 0], in=0, p20q=on}
      mask prompts: p2q "Power Rating [MVA]"; p3q "Active Power [p.u.]"; p4_5q "Max and Min Power Supply [p.u.  p.u.]"; p7_8_9q "Cost = a + b*P + c*P^2 [$/h, $/MWh, $/(MW)^2 h]"; p10_11_12q "Cost = a + b*Q + c*Q^2 [$/h, $/MVArh, $/(MVAr)^2 h]"; p13q "Allow Unit Commitment"; p14q "Tie Breaking Cost [$/h]"; p15q "Loss participation factor"; p16_17q "Reactive power limits Qmax and Qmin [p.u. p.u.]"; p18_19q "Up and down congestion costs [$/h $/h]"; in "Number of Input Signals"; p20q "Connected"
      mask help: This block defines a PV bus for bifurcation and market studies:
      mask init:
      | fm_inout;
      | [x,y] = fm_draw('circle');
      | [xs,ys] = fm_draw('$');
      mask StyleString: edit,edit,edit,edit,edit,checkbox,edit,edit,edit,edit,popup(0|1|2),checkbox
      mask CallbackString: |||||||||||fm_block
      mask Display:
      | plot(x,y)
      | color('blue')
      | plot(xs,ys)
  Sup122d : PMComponent  Tag=PSATblock  Description=OPF & CPF  Orientation=down  PhysicalDomain=psatdomain  LeftPortType=p1  RightPortType=p1  RConnTagsString=__newr0  mask(Supply){p2q=100, p3q=0.5, p4_5q=[0.5  0], p7_8_9q=[0.00  1  0.00], p10_11_12q=[0.00  0.00  0.00], p13q=off, p14q=0, p15q=1, p16_17q=[0.16  -0.1], p18_19q=[0 0], in=0, p20q=on}
      mask prompts: p2q "Power Rating [MVA]"; p3q "Active Power [p.u.]"; p4_5q "Max and Min Power Supply [p.u.  p.u.]"; p7_8_9q "Cost = a + b*P + c*P^2 [$/h, $/MWh, $/(MW)^2 h]"; p10_11_12q "Cost = a + b*Q + c*Q^2 [$/h, $/MVArh, $/(MVAr)^2 h]"; p13q "Allow Unit Commitment"; p14q "Tie Breaking Cost [$/h]"; p15q "Loss participation factor"; p16_17q "Reactive power limits Qmax and Qmin [p.u. p.u.]"; p18_19q "Up and down congestion costs [$/h $/h]"; in "Number of Input Signals"; p20q "Connected"
      mask help: This block defines a PV bus for bifurcation and market studies:
      mask init:
      | fm_inout;
      | [x,y] = fm_draw('circle');
      | [xs,ys] = fm_draw('$');
      mask StyleString: edit,edit,edit,edit,edit,checkbox,edit,edit,edit,edit,popup(0|1|2),checkbox
      mask CallbackString: |||||||||||fm_block
      mask Display:
      | plot(x,y)
      | color('blue')
      | plot(xs,ys)
  Sup122e : PMComponent  Tag=PSATblock  Description=OPF & CPF  Orientation=down  PhysicalDomain=psatdomain  LeftPortType=p1  RightPortType=p1  RConnTagsString=__newr0  mask(Supply){p2q=100, p3q=0.5, p4_5q=[0.5  0], p7_8_9q=[0.00  1  0.00], p10_11_12q=[0.00  0.00  0.00], p13q=off, p14q=0, p15q=1, p16_17q=[0.16  -0.1], p18_19q=[0 0], in=0, p20q=on}
      mask prompts: p2q "Power Rating [MVA]"; p3q "Active Power [p.u.]"; p4_5q "Max and Min Power Supply [p.u.  p.u.]"; p7_8_9q "Cost = a + b*P + c*P^2 [$/h, $/MWh, $/(MW)^2 h]"; p10_11_12q "Cost = a + b*Q + c*Q^2 [$/h, $/MVArh, $/(MVAr)^2 h]"; p13q "Allow Unit Commitment"; p14q "Tie Breaking Cost [$/h]"; p15q "Loss participation factor"; p16_17q "Reactive power limits Qmax and Qmin [p.u. p.u.]"; p18_19q "Up and down congestion costs [$/h $/h]"; in "Number of Input Signals"; p20q "Connected"
      mask help: This block defines a PV bus for bifurcation and market studies:
      mask init:
      | fm_inout;
      | [x,y] = fm_draw('circle');
      | [xs,ys] = fm_draw('$');
      mask StyleString: edit,edit,edit,edit,edit,checkbox,edit,edit,edit,edit,popup(0|1|2),checkbox
      mask CallbackString: |||||||||||fm_block
      mask Display:
      | plot(x,y)
      | color('blue')
      | plot(xs,ys)
  Sup122f : PMComponent  Tag=PSATblock  Description=OPF & CPF  Orientation=down  PhysicalDomain=psatdomain  LeftPortType=p1  RightPortType=p1  RConnTagsString=__newr0  mask(Supply){p2q=100, p3q=0.5, p4_5q=[0.5  0], p7_8_9q=[0.00  1  0.00], p10_11_12q=[0.00  0.00  0.00], p13q=off, p14q=0, p15q=1, p16_17q=[0.16  -0.1], p18_19q=[0 0], in=0, p20q=on}
      mask prompts: p2q "Power Rating [MVA]"; p3q "Active Power [p.u.]"; p4_5q "Max and Min Power Supply [p.u.  p.u.]"; p7_8_9q "Cost = a + b*P + c*P^2 [$/h, $/MWh, $/(MW)^2 h]"; p10_11_12q "Cost = a + b*Q + c*Q^2 [$/h, $/MVArh, $/(MVAr)^2 h]"; p13q "Allow Unit Commitment"; p14q "Tie Breaking Cost [$/h]"; p15q "Loss participation factor"; p16_17q "Reactive power limits Qmax and Qmin [p.u. p.u.]"; p18_19q "Up and down congestion costs [$/h $/h]"; in "Number of Input Signals"; p20q "Connected"
      mask help: This block defines a PV bus for bifurcation and market studies:
      mask init:
      | fm_inout;
      | [x,y] = fm_draw('circle');
      | [xs,ys] = fm_draw('$');
      mask StyleString: edit,edit,edit,edit,edit,checkbox,edit,edit,edit,edit,popup(0|1|2),checkbox
      mask CallbackString: |||||||||||fm_block
      mask Display:
      | plot(x,y)
      | color('blue')
      | plot(xs,ys)
  Sup123 : PMComponent  Tag=PSATblock  Description=OPF & CPF  Orientation=left  PhysicalDomain=psatdomain  LeftPortType=p1  RightPortType=p1  RConnTagsString=__newr0  mask(Supply){p2q=100, p3q=1.55, p4_5q=[1.55  0.5425], p7_8_9q=[0.0109*100  9.5369  0.5586/100], p10_11_12q=[0.00  0.00  0.00], p13q=off, p14q=0, p15q=1, p16_17q=[0.8  -0.5], p18_19q=[0 0], in=0, p20q=on}
      mask prompts: p2q "Power Rating [MVA]"; p3q "Active Power [p.u.]"; p4_5q "Max and Min Power Supply [p.u.  p.u.]"; p7_8_9q "Cost = a + b*P + c*P^2 [$/h, $/MWh, $/(MW)^2 h]"; p10_11_12q "Cost = a + b*Q + c*Q^2 [$/h, $/MVArh, $/(MVAr)^2 h]"; p13q "Allow Unit Commitment"; p14q "Tie Breaking Cost [$/h]"; p15q "Loss participation factor"; p16_17q "Reactive power limits Qmax and Qmin [p.u. p.u.]"; p18_19q "Up and down congestion costs [$/h $/h]"; in "Number of Input Signals"; p20q "Connected"
      mask help: This block defines a PV bus for bifurcation and market studies:
      mask init:
      | fm_inout;
      | [x,y] = fm_draw('circle');
      | [xs,ys] = fm_draw('$');
      mask StyleString: edit,edit,edit,edit,edit,checkbox,edit,edit,edit,edit,popup(0|1|2),checkbox
      mask CallbackString: |||||||||||fm_block
      mask Display:
      | plot(x,y)
      | color('blue')
      | plot(xs,ys)
  Sup8 : PMComponent  Tag=PSATblock  Description=OPF & CPF  Orientation=left  PhysicalDomain=psatdomain  LeftPortType=p1  RightPortType=p1  RConnTagsString=__newr0  mask(Supply){p2q=100, p3q=1.55, p4_5q=[1.55  0.5425], p7_8_9q=[0.0109*100  9.5369  0.5586/100], p10_11_12q=[0.00  0.00  0.00], p13q=off, p14q=0, p15q=1, p16_17q=[0.8  -0.5], p18_19q=[0 0], in=0, p20q=on}
      mask prompts: p2q "Power Rating [MVA]"; p3q "Active Power [p.u.]"; p4_5q "Max and Min Power Supply [p.u.  p.u.]"; p7_8_9q "Cost = a + b*P + c*P^2 [$/h, $/MWh, $/(MW)^2 h]"; p10_11_12q "Cost = a + b*Q + c*Q^2 [$/h, $/MVArh, $/(MVAr)^2 h]"; p13q "Allow Unit Commitment"; p14q "Tie Breaking Cost [$/h]"; p15q "Loss participation factor"; p16_17q "Reactive power limits Qmax and Qmin [p.u. p.u.]"; p18_19q "Up and down congestion costs [$/h $/h]"; in "Number of Input Signals"; p20q "Connected"
      mask help: This block defines a PV bus for bifurcation and market studies:
      mask init:
      | fm_inout;
      | [x,y] = fm_draw('circle');
      | [xs,ys] = fm_draw('$');
      mask StyleString: edit,edit,edit,edit,edit,checkbox,edit,edit,edit,edit,popup(0|1|2),checkbox
      mask CallbackString: |||||||||||fm_block
      mask Display:
      | plot(x,y)
      | color('blue')
      | plot(xs,ys)
  Sup9 : PMComponent  Tag=PSATblock  Description=OPF & CPF  Orientation=left  PhysicalDomain=psatdomain  LeftPortType=p1  RightPortType=p1  RConnTagsString=__newr0  mask(Supply){p2q=100, p3q=3.50, p4_5q=[3.50  1.40], p7_8_9q=[0.0164*100  9.5856  0.3152/100], p10_11_12q=[0.00  0.00  0.00], p13q=off, p14q=0, p15q=1, p16_17q=[1.5  -0.25], p18_19q=[0 0], in=0, p20q=on}
      mask prompts: p2q "Power Rating [MVA]"; p3q "Active Power [p.u.]"; p4_5q "Max and Min Power Supply [p.u.  p.u.]"; p7_8_9q "Cost = a + b*P + c*P^2 [$/h, $/MWh, $/(MW)^2 h]"; p10_11_12q "Cost = a + b*Q + c*Q^2 [$/h, $/MVArh, $/(MVAr)^2 h]"; p13q "Allow Unit Commitment"; p14q "Tie Breaking Cost [$/h]"; p15q "Loss participation factor"; p16_17q "Reactive power limits Qmax and Qmin [p.u. p.u.]"; p18_19q "Up and down congestion costs [$/h $/h]"; in "Number of Input Signals"; p20q "Connected"
      mask help: This block defines a PV bus for bifurcation and market studies:
      mask init:
      | fm_inout;
      | [x,y] = fm_draw('circle');
      | [xs,ys] = fm_draw('$');
      mask StyleString: edit,edit,edit,edit,edit,checkbox,edit,edit,edit,edit,popup(0|1|2),checkbox
      mask CallbackString: |||||||||||fm_block
      mask Display:
      | plot(x,y)
      | color('blue')
      | plot(xs,ys)
  connections:
  Sup113c/RConn1 -- Bus113/LConn4
  Sup113b/RConn1 -- Bus113/LConn3
  Sup107c/RConn1 -- Bus107/LConn4
  Sup107b/RConn1 -- Bus107/LConn3
  Sup107a/RConn1 -- Bus107/LConn2
  Gen107/RConn1 -- Bus107/LConn1
  Sup115f/RConn1 -- Bus115/LConn8
  Sup115e/RConn1 -- Bus115/LConn7
  Sup115d/RConn1 -- Bus115/LConn6
  Sup115c/RConn1 -- Bus115/LConn5
  Sup115b/RConn1 -- Bus115/LConn4
  A25_1/RConn1 -- Bus115/LConn9
  A25_2/RConn1 -- Bus115/LConn10
  Bus116/RConn3 -- Dem116/LConn1
  Bus116/RConn2 -- A24/LConn1
  Sup9/RConn1 -- Bus123/LConn4
  Sup8/RConn1 -- Bus123/LConn3
  A22/RConn1 -- Bus123/LConn5
  Sup122f/RConn1 -- Bus122/LConn8
  Sup122e/RConn1 -- Bus122/LConn7
  Sup122d/RConn1 -- Bus122/LConn6
  Sup122c/RConn1 -- Bus122/LConn5
  Sup122b/RConn1 -- Bus122/LConn4
  Sup113a/RConn1 -- Bus113/LConn2
  Gen113/RConn1 -- Bus113/LConn1
  Sup102d/RConn1 -- Bus102/LConn5
  Sup101d/RConn1 -- Bus101/LConn5
  Sup101c/RConn1 -- Bus101/LConn4
  Sup101b/RConn1 -- Bus101/LConn3
  Sup101a/RConn1 -- Bus101/LConn2
  Gen101/RConn1 -- Bus101/LConn1
  A05/RConn1 -- Bus106/LConn2
  Bus105/RConn2 -- Dem105/LConn1
  Bus105/RConn1 -- Load105/LConn1
  A03/RConn1 -- Bus105/LConn1
  A09/RConn1 -- Bus105/LConn2
  A04/RConn1 -- Bus104/LConn2
  Bus101/RConn5 -- A01/LConn1
  Bus107/RConn2 -- Dem107/LConn1
  Bus107/RConn3 -- Load107/LConn1
  A11/RConn1 -- Bus108/LConn3
  Bus107/RConn1 -- A11/LConn1
  A02/RConn1 -- Bus103/LConn3
  A06/RConn1 -- Bus103/LConn2
  A1/LConn1 -- Bus103/LConn1
  Bus103/RConn1 -- Dem103/LConn1
  Bus103/RConn2 -- Load103/LConn1
  Bus101/RConn4 -- A03/LConn1
  Bus101/RConn3 -- Load101/LConn1
  Bus101/RConn2 -- Dem101/LConn1
  Bus101/RConn1 -- A02/LConn1
  Bus104/RConn2 -- Load104/LConn1
  Bus104/RConn1 -- Dem104/LConn1
  Bus110/RConn3 -- A09/LConn1
  Bus110/RConn2 -- Load110/LConn1
  A08/RConn1 -- Bus104/LConn1
  Bus109/RConn4 -- Dem109/LConn1
  Bus109/RConn1 -- A06/LConn1
  Bus109/RConn3 -- Load109/LConn1
  Bus109/RConn2 -- A08/LConn1
  Bus110/RConn1 -- Dem110/LConn1
  Bus109/RConn5 -- A12_1/LConn1
  Bus108/RConn2 -- Dem108/LConn1
  Bus108/RConn1 -- Load108/LConn1
  A12_1/RConn1 -- Bus108/LConn2
  A13_2/RConn1 -- Bus108/LConn1
  Bus110/RConn4 -- A13_2/LConn1
  Bus106/RConn2 -- Dem106/LConn1
  Bus106/RConn1 -- Load106/LConn1
  Bus106/RConn3 -- Shunt106/LConn1
  A10/RConn1 -- Bus106/LConn1
  Bus110/RConn5 -- A10/LConn1
  A5/LConn1 -- Bus110/LConn1
  A3/LConn1 -- Bus109/LConn2
  A4/LConn1 -- Bus110/LConn2
  A2/LConn1 -- Bus109/LConn1
  Bus112/RConn1 -- A3/RConn1
  Bus112/RConn2 -- A4/RConn1
  A21/RConn1 -- Bus112/LConn1
  Bus123/RConn3 -- A21/LConn1
  A20/RConn1 -- Bus112/LConn2
  Bus113/RConn5 -- A20/LConn1
  Bus113/RConn1 -- A22/LConn1
  Bus113/RConn3 -- Load113/LConn1
  Bus113/RConn4 -- A18/LConn1
  Bus113/RConn2 -- Dem113/LConn1
  A18/RConn1 -- Bus111/LConn2
  Bus111/RConn1 -- A2/RConn1
  Bus111/RConn2 -- A5/RConn1
  A19/RConn1 -- Bus111/LConn1
  Bus114/RConn3 -- A19/LConn1
  Bus124/RConn1 -- A1/RConn1
  A26/RConn1 -- Bus124/LConn1
  Bus115/RConn3 -- A26/LConn1
  Bus114/RConn2 -- Dem114/LConn1
  Bus114/RConn1 -- Load114/LConn1
  A23/RConn1 -- Bus114/LConn1
  Bus116/RConn4 -- A23/LConn1
  Gen114/RConn1 -- Bus114/LConn2
  Bus115/RConn2 -- Dem115/LConn1
  Bus119/RConn5 -- Dem119/LConn1
  Bus120/RConn2 -- Dem120/LConn1
  Bus118/RConn1 -- Dem118/LConn1
  Bus118/RConn3 -- A29/LConn1
  Bus118/RConn4 -- A31_2/LConn1
  Bus118/RConn5 -- A31_1/LConn1
  Sup115a/RConn1 -- Bus115/LConn2
  A24/RConn1 -- Bus115/LConn3
  Sup116/RConn1 -- Bus116/LConn3
  A28/RConn1 -- Bus116/LConn4
  Sup123/RConn1 -- Bus123/LConn2
  Sup122a/RConn1 -- Bus122/LConn3
  Sup121/RConn1 -- Bus121/LConn4
  Sup118/RConn1 -- Bus118/LConn2
  Bus115/RConn1 -- Load115/LConn1
  Gen115/RConn1 -- Bus115/LConn1
  Bus119/RConn4 -- Load119/LConn1
  Bus120/RConn1 -- Load120/LConn1
  Bus119/RConn2 -- A32_1/LConn1
  Bus119/RConn3 -- A32_2/LConn1
  Bus119/RConn1 -- A28/LConn1
  Gen116/RConn1 -- Bus116/LConn2
  A32_2/RConn1 -- Bus120/LConn1
  A32_1/RConn1 -- Bus120/LConn2
  A33_1/RConn1 -- Bus120/LConn3
  A33_2/RConn1 -- Bus120/LConn4
  Bus123/RConn2 -- A33_2/LConn1
  Bus123/RConn1 -- A33_1/LConn1
  Gen123/RConn1 -- Bus123/LConn1
  Bus116/RConn1 -- Load116/LConn1
  A27/RConn1 -- Bus116/LConn1
  Bus117/RConn1 -- A27/LConn1
  Bus121/RConn2 -- A25_2/LConn1
  Bus121/RConn1 -- A25_1/LConn1
  A30/RConn1 -- Bus117/LConn2
  Bus122/RConn1 -- A30/LConn1
  Gen122/RConn1 -- Bus122/LConn2
  A34/RConn1 -- Bus122/LConn1
  Bus121/RConn3 -- A34/LConn1
  A31_2/RConn1 -- Bus121/LConn1
  A31_1/RConn1 -- Bus121/LConn2
  Gen121/RConn1 -- Bus121/LConn3
  Gen118/RConn1 -- Bus118/LConn1
  Bus118/RConn2 -- Load118/LConn1
  A29/RConn1 -- Bus117/LConn1
  A05/LConn1 -- Bus102/RConn5
  Bus102/RConn4 -- Load102/LConn1
  Dem102/LConn1 -- Bus102/RConn3
  A04/LConn1 -- Bus102/RConn2
  A01/RConn1 -- Bus102/RConn1
  Gen102/RConn1 -- Bus102/LConn1
  Sup102a/RConn1 -- Bus102/LConn2
  Sup102c/RConn1 -- Bus102/LConn4
  Sup102b/RConn1 -- Bus102/LConn3
